simulink model "UPQC_model"  (R2020b)
settings: Solver=FixedStepAuto  StartTime=0.0  StopTime=Tsim  FixedStep=Tsample  MaxStep=Tsample  RelTol=1e-3
values from neighbouring files (symbols this model uses):
  C_parallel_Series = zeros(1,4)    [Netzmodell_Ini_DL.m]    (also in workspace_Ini.mat = [1e-05 1e-05 1e-05 0])
  C_parallel_Shunt = zeros(1,4)    [Netzmodell_Ini_DL.m]    (also in workspace_Ini.mat = [1e-05 1e-05 1e-05 0])
  CC_Ki = 5    [Netzmodell_Ini_DL.m]    (also in workspace_Ini.mat)
  CC_Ki_geg = 5    [Netzmodell_Ini_DL.m]    (also in workspace_Ini.mat)
  CC_Kp = 10    [Netzmodell_Ini_DL.m]    (also in workspace_Ini.mat)
  CC_Kp_geg = 10    [Netzmodell_Ini_DL.m]    (also in workspace_Ini.mat)
  CC_OS =     [workspace_Ini.mat]
  Czk = Szenario.Czk*u    [Netzmodell_Ini_DL.m]    (also in workspace_Ini.mat = 0.003)
  fak_RVC = Szenario.fak_RVC    [Netzmodell_Ini_DL.m]    (also in workspace_Ini.mat = [1 1 1])
  fak_Uns = [1; 1; 1]    [Netzmodell_Ini_DL.m]    (also in workspace_Ini.mat = [1 1 1])
  Flicker_Schaltzeitpunkte_L1 = Schaltzeitpunkte(1,:)    [Netzmodell_Ini_DL.m]    (also in workspace_Ini.mat = 10.5)
  Flicker_Schaltzeitpunkte_L2 = Schaltzeitpunkte(2,:)    [Netzmodell_Ini_DL.m]    (also in workspace_Ini.mat = 10.5)
  Flicker_Schaltzeitpunkte_L3 = Schaltzeitpunkte(3,:)    [Netzmodell_Ini_DL.m]    (also in workspace_Ini.mat = 10.5)
  fs = [f_nom; f_nom; f_nom]    [Netzmodell_Ini_DL.m]    (also in workspace_Ini.mat = [50 50 50])
  fsw = Szenario.fsw*k    [Netzmodell_Ini_DL.m]    (also in workspace_Ini.mat = 20000)
  I_Basis_Ober_L1 = I_Basis_Ober(1)    [Netzmodell_Ini_DL.m]    (also in workspace_Ini.mat = 0)
  I_Basis_Ober_L2 = I_Basis_Ober(2)    [Netzmodell_Ini_DL.m]    (also in workspace_Ini.mat = 0)
  I_Basis_Ober_L3 = I_Basis_Ober(3)    [Netzmodell_Ini_DL.m]    (also in workspace_Ini.mat = 0)
  I_relativ_Ober_L1 = Szenario.I_relativ_Ober_L1    [Netzmodell_Ini_DL.m]    (also in workspace_Ini.mat = [0 100 0 100 100 0 100 100 0 0 0 0 ... (50 elements, 1x50)])
  I_relativ_Ober_L2 = Szenario.I_relativ_Ober_L2    [Netzmodell_Ini_DL.m]    (also in workspace_Ini.mat = [0 100 0 100 100 0 100 100 0 0 0 0 ... (50 elements, 1x50)])
  I_relativ_Ober_L3 = Szenario.I_relativ_Ober_L3    [Netzmodell_Ini_DL.m]    (also in workspace_Ini.mat = [0 100 0 100 100 0 100 100 0 0 0 0 ... (50 elements, 1x50)])
  L_Ausgang_Series = zeros(1,4)    [Netzmodell_Ini_DL.m]    (also in workspace_Ini.mat = [0.00093 0.00093 0.00093 0.00093])
  L_Ausgang_Shunt = zeros(1,4)    [Netzmodell_Ini_DL.m]    (also in workspace_Ini.mat = [0.00093 0.00093 0.00093 0.00093])
  L_Eingang_Series = zeros(1,4)    [Netzmodell_Ini_DL.m]    (also in workspace_Ini.mat = [0.00085 0.00085 0.00085 0.00085])
  L_Eingang_Shunt = zeros(1,4)    [Netzmodell_Ini_DL.m]    (also in workspace_Ini.mat = [0.00085 0.00085 0.00085 0.00085])
  Ls_in = 52.2*u/10    (= 5.22e-06)    [Netzmodell_Ini_DL.m]    (also in workspace_Ini.mat)
  Ltrans = Szenario.Ltrans*m    [Netzmodell_Ini_DL.m]    (also in workspace_Ini.mat = 0.000256)
  OS_off = 6    [Netzmodell_Ini_DL.m]    (also in workspace_Ini.mat)
  OS_on = 1    [Netzmodell_Ini_DL.m]    (also in workspace_Ini.mat)
  Phi_Ober_L1 = Phi_Ober(1)    [Netzmodell_Ini_DL.m]    (also in workspace_Ini.mat = 0)
  Phi_Ober_L2 = Phi_Ober(2)    [Netzmodell_Ini_DL.m]    (also in workspace_Ini.mat = -120)
  Phi_Ober_L3 = Phi_Ober(3)    [Netzmodell_Ini_DL.m]    (also in workspace_Ini.mat = 120)
  Phis = [0; -120; 120]    [Netzmodell_Ini_DL.m]    (also in workspace_Ini.mat = [0 -120 120])
  Pl_Flicker = Pl_Flicker*k    [Netzmodell_Ini_DL.m]    (also in workspace_Ini.mat = [5000 5000 5000])
  Pl_Grund = Szenario.Pl_Grund *k    [Netzmodell_Ini_DL.m]    (also in workspace_Ini.mat = [5 5 5])
  Pl_RVC = Pl_RVC*k    [Netzmodell_Ini_DL.m]    (also in workspace_Ini.mat = [10000 10000 10000])
  Pl_Uns = Pl_Uns*k    [Netzmodell_Ini_DL.m]    (also in workspace_Ini.mat = [25000 10 10])
  Ql_ind_Flicker = Ql_ind_Flicker*k    [Netzmodell_Ini_DL.m]    (also in workspace_Ini.mat = [0 0 0])
  Ql_ind_Grund = Szenario.Ql_ind_Grund*k    [Netzmodell_Ini_DL.m]    (also in workspace_Ini.mat = [0 0 0])
  Ql_ind_RVC = Szenario.Ql_ind_RVC*k    [Netzmodell_Ini_DL.m]    (also in workspace_Ini.mat = [0 0 0])
  Ql_ind_Uns = Ql_ind_Uns*k    [Netzmodell_Ini_DL.m]    (also in workspace_Ini.mat = [0 0 0])
  Ql_kap_Flicker = Ql_kap_Flicker*k    [Netzmodell_Ini_DL.m]    (also in workspace_Ini.mat = [0 0 0])
  Ql_kap_Grund = Szenario.Ql_kap_Grund*k    [Netzmodell_Ini_DL.m]    (also in workspace_Ini.mat = [0 0 0])
  Ql_kap_RVC = Szenario.Ql_kap_RVC*k    [Netzmodell_Ini_DL.m]    (also in workspace_Ini.mat = [0 0 0])
  Ql_kap_Uns = Ql_kap_Uns*k    [Netzmodell_Ini_DL.m]    (also in workspace_Ini.mat = [0 0 0])
  R_Ausgang_Series = zeros(1,4)    [Netzmodell_Ini_DL.m]    (also in workspace_Ini.mat = [0.1 0.1 0.1 0.1])
  R_Ausgang_Shunt = zeros(1,4)    [Netzmodell_Ini_DL.m]    (also in workspace_Ini.mat = [0.1 0.1 0.1 0.1])
  R_Eingang_Series = zeros(1,4)    [Netzmodell_Ini_DL.m]    (also in workspace_Ini.mat = [0.1 0.1 0.1 0.1])
  R_Eingang_Shunt = zeros(1,4)    [Netzmodell_Ini_DL.m]    (also in workspace_Ini.mat = [0.1 0.1 0.1 0.1])
  R_parallel_Series = zeros(1,4)    [Netzmodell_Ini_DL.m]    (also in workspace_Ini.mat = [13 13 13 0])
  R_parallel_Shunt = zeros(1,4)    [Netzmodell_Ini_DL.m]    (also in workspace_Ini.mat = [13 13 13 0])
  R_ZK_Belastung = 20    [Netzmodell_Ini_DL.m]    (also in workspace_Ini.mat)
  Rs_in = 5.2*m/10    (= 0.00052)    [Netzmodell_Ini_DL.m]    (also in workspace_Ini.mat)
  Rtrans = Szenario.Rtrans    [Netzmodell_Ini_DL.m]    (also in workspace_Ini.mat = 0.206)
  RVC_L1_on_off_Zeitpunkte = Szenario.RVC_L1_on_off_Zeitpunkte    [Netzmodell_Ini_DL.m]    (also in workspace_Ini.mat = [10.5 40 10 11 12 13 14 15])
  RVC_L2_on_off_Zeitpunkte = Szenario.RVC_L2_on_off_Zeitpunkte    [Netzmodell_Ini_DL.m]    (also in workspace_Ini.mat = [10.5 40 10 11 12 13 14 15])
  RVC_L3_on_off_Zeitpunkte = Szenario.RVC_L3_on_off_Zeitpunkte    [Netzmodell_Ini_DL.m]    (also in workspace_Ini.mat = [10.5 40 10 11 12 13 14 15])
  RVC_off = 20.5    [Netzmodell_Ini_DL.m]    (also in workspace_Ini.mat)
  RVC_on = 20    [Netzmodell_Ini_DL.m]    (also in workspace_Ini.mat)
  RVC_val = [0.8,0.8,0.8]    [Netzmodell_Ini_DL.m]    (also in workspace_Ini.mat = [0.8 0.8 0.8])
  strans = Szenario.strans    [Netzmodell_Ini_DL.m]    (also in workspace_Ini.mat = 0.25)
  t_breaker_series = tacts    [Netzmodell_Ini_DL.m]    (also in workspace_Ini.mat = 0.5)
  tact = Szenario.tact    [Netzmodell_Ini_DL.m]    (also in workspace_Ini.mat = 0.5)
  tact_OS_Regler = Szenario.tact_OS_Regler    [Netzmodell_Ini_DL.m]    (also in workspace_Ini.mat = 0.5)
  tact_QU = 10    [Netzmodell_Ini_DL.m]    (also in workspace_Ini.mat)
  tacts = Szenario.tacts    [Netzmodell_Ini_DL.m]    (also in workspace_Ini.mat = 0.5)
  Tsample = Szenario.Tsample    [Netzmodell_Ini_DL.m]    (also in workspace_Ini.mat = 5e-06)
  Uns_L1_on_off_Zeitpunkte = Szenario.Uns_L1_on_off_Zeitpunkte    [Netzmodell_Ini_DL.m]    (also in workspace_Ini.mat = [1 6 10 11 12 13 14 15])
  Uns_L2_on_off_Zeitpunkte = Szenario.Uns_L2_on_off_Zeitpunkte    [Netzmodell_Ini_DL.m]    (also in workspace_Ini.mat = [10 30 10 11 12 13 14 15])
  Uns_L3_on_off_Zeitpunkte = Szenario.Uns_L3_on_off_Zeitpunkte    [Netzmodell_Ini_DL.m]    (also in workspace_Ini.mat = [10 30 10 11 12 13 14 15])
  Us = [Us_Amp; Us_Amp; Us_Amp]    [Netzmodell_Ini_DL.m]    (also in workspace_Ini.mat = [326.598632371 326.598632371 326.598632371])
  Us_Amp = sqrt(2)*400/sqrt(3)    [Netzmodell_Ini_DL.m]    (also in workspace_Ini.mat = 326.598632371)
  VC_Ki_gegen = 30    [Netzmodell_Ini_DL.m]    (also in workspace_Ini.mat)
  VC_Ki_gegen_shunt = 15    [Netzmodell_Ini_DL.m]    (also in workspace_Ini.mat)
  VC_Ki_mit = 5    [Netzmodell_Ini_DL.m]    (also in workspace_Ini.mat)
  VC_Kp_gegen = 5    [workspace_Ini.mat]
  VC_Kp_gegen_shunt = 2    [Netzmodell_Ini_DL.m]    (also in workspace_Ini.mat)
  VC_Kp_mit = 10    [Netzmodell_Ini_DL.m]    (also in workspace_Ini.mat)
  VC_ZK_Ki = 5    [Netzmodell_Ini_DL.m]    (also in workspace_Ini.mat)
  VC_ZK_Kp = 0.5    [Netzmodell_Ini_DL.m]    (also in workspace_Ini.mat)
  Vielfache_Ober_L1 = Szenario.Vielfache_Ober_L1    [Netzmodell_Ini_DL.m]    (also in workspace_Ini.mat = [1 2 3 4 5 6 7 8 9 10 11 12 ... (50 elements, 1x50)])
  Vielfache_Ober_L2 = Szenario.Vielfache_Ober_L2    [Netzmodell_Ini_DL.m]    (also in workspace_Ini.mat = [1 2 3 4 5 6 7 8 9 10 11 12 ... (50 elements, 1x50)])
  Vielfache_Ober_L3 = Szenario.Vielfache_Ober_L3    [Netzmodell_Ini_DL.m]    (also in workspace_Ini.mat = [1 2 3 4 5 6 7 8 9 10 11 12 ... (50 elements, 1x50)])
  ZK_Belastung_off = 100    [Netzmodell_Ini_DL.m]    (also in workspace_Ini.mat)
  ZK_Belastung_on = 100    [Netzmodell_Ini_DL.m]    (also in workspace_Ini.mat)
  Zwischenkreisspannung = 700    [Netzmodell_Ini_DL.m]    (also in workspace_Ini.mat)
undefined symbols (not defined in the file or in its folder): LAusgang, RReiheL3
libraries: powerlib x221, powerlib_meascontrol x80, pid_lib x23, eeTransforms x4, eePwmGeneratorTwoLevel x2, dspstat3 x1
(part 11 of 16)

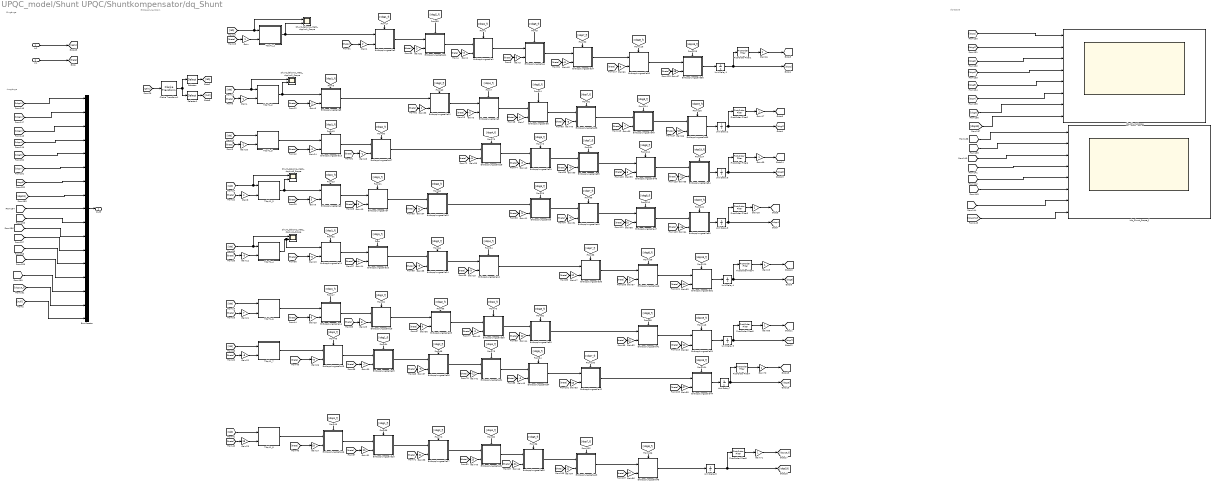
== system UPQC_model/Shunt UPQC/Shuntkompensator/dq_Shunt ==
  note: Entkopplung Strom
  note: Eingänge
  note: Ausgänge
  note: dq-Scope
  In2 : Inport
  In1 : Inport  Port=2
  Bus Creator : BusCreator  Inputs=17
  Clarke Transform1 : eeTransforms/Clarke Transform  PowerInvariant=off
      settings: SourceProductBaseCode=PS
  Entkopplungszelle1 : Subsystem
      settings: PortSchema="{\"entries\":[{\"content\":{\"sides\":[{\"content\":{\"connectorIds\":[\"In1\",\"In2\"]},\"type\":\"ConnectorPlacement.EquallySpacedRectSide\",\"uuid\":\"e8e24803-2fc0-483c-82f9-6ee33f65ebd9\"},{\"content\":{\"connectorIds\":[\"Out1\"],\"side\":\"RIGHT\"},\"type\":\"ConnectorPlacement.EquallySpacedRectSide\",\"uuid\":\"e11e5831-ab5e-42bb-bd0b-63825273f403\"},{\"content\":{\"connectorIds\":[\"In3\"],\"side\":\"TOP\"},\"type\":\"ConnectorPlacement.EquallySpacedRectSide\",\"uuid\":\"2b39bd07-2b6e-4e89-bb54-1321cea2c793\"},{\"content\":{\"connectorIds\":[],\"side\":\"HIDDEN\"},\"type\":\"ConnectorPlacement.EquallySpacedRectSide\",\"uuid\":\"a99c5943-5af0-4d11-8875-695bd24f17f4\"}]},\"type\":\"ConnectorPlacement.EquallySpacedConnector\",\"uuid\":\"a2a714db-f067-4e0e-8919-f68d1dab84ba\"}],\"packageUris\":[\"http://schema.mathworks.com/mf0/Connector/R2020b\"],\"version\":\"1.0\"}"
  Entkopplungszelle10 : Subsystem
      settings: PortSchema="{\"entries\":[{\"content\":{\"sides\":[{\"content\":{\"connectorIds\":[\"In1\",\"In2\"]},\"type\":\"ConnectorPlacement.EquallySpacedRectSide\",\"uuid\":\"e8e24803-2fc0-483c-82f9-6ee33f65ebd9\"},{\"content\":{\"connectorIds\":[\"Out1\"],\"side\":\"RIGHT\"},\"type\":\"ConnectorPlacement.EquallySpacedRectSide\",\"uuid\":\"e11e5831-ab5e-42bb-bd0b-63825273f403\"},{\"content\":{\"connectorIds\":[\"In3\"],\"side\":\"TOP\"},\"type\":\"ConnectorPlacement.EquallySpacedRectSide\",\"uuid\":\"2b39bd07-2b6e-4e89-bb54-1321cea2c793\"},{\"content\":{\"connectorIds\":[],\"side\":\"HIDDEN\"},\"type\":\"ConnectorPlacement.EquallySpacedRectSide\",\"uuid\":\"a99c5943-5af0-4d11-8875-695bd24f17f4\"}]},\"type\":\"ConnectorPlacement.EquallySpacedConnector\",\"uuid\":\"a2a714db-f067-4e0e-8919-f68d1dab84ba\"}],\"packageUris\":[\"http://schema.mathworks.com/mf0/Connector/R2020b\"],\"version\":\"1.0\"}"
  Entkopplungszelle11 : Subsystem
      settings: PortSchema="{\"entries\":[{\"content\":{\"sides\":[{\"content\":{\"connectorIds\":[\"In1\",\"In2\"]},\"type\":\"ConnectorPlacement.EquallySpacedRectSide\",\"uuid\":\"e8e24803-2fc0-483c-82f9-6ee33f65ebd9\"},{\"content\":{\"connectorIds\":[\"Out1\"],\"side\":\"RIGHT\"},\"type\":\"ConnectorPlacement.EquallySpacedRectSide\",\"uuid\":\"e11e5831-ab5e-42bb-bd0b-63825273f403\"},{\"content\":{\"connectorIds\":[\"In3\"],\"side\":\"TOP\"},\"type\":\"ConnectorPlacement.EquallySpacedRectSide\",\"uuid\":\"2b39bd07-2b6e-4e89-bb54-1321cea2c793\"},{\"content\":{\"connectorIds\":[],\"side\":\"HIDDEN\"},\"type\":\"ConnectorPlacement.EquallySpacedRectSide\",\"uuid\":\"a99c5943-5af0-4d11-8875-695bd24f17f4\"}]},\"type\":\"ConnectorPlacement.EquallySpacedConnector\",\"uuid\":\"a2a714db-f067-4e0e-8919-f68d1dab84ba\"}],\"packageUris\":[\"http://schema.mathworks.com/mf0/Connector/R2020b\"],\"version\":\"1.0\"}"
  Entkopplungszelle12 : Subsystem
      settings: PortSchema="{\"entries\":[{\"content\":{\"sides\":[{\"content\":{\"connectorIds\":[\"In1\",\"In2\"]},\"type\":\"ConnectorPlacement.EquallySpacedRectSide\",\"uuid\":\"e8e24803-2fc0-483c-82f9-6ee33f65ebd9\"},{\"content\":{\"connectorIds\":[\"Out1\"],\"side\":\"RIGHT\"},\"type\":\"ConnectorPlacement.EquallySpacedRectSide\",\"uuid\":\"e11e5831-ab5e-42bb-bd0b-63825273f403\"},{\"content\":{\"connectorIds\":[\"In3\"],\"side\":\"TOP\"},\"type\":\"ConnectorPlacement.EquallySpacedRectSide\",\"uuid\":\"2b39bd07-2b6e-4e89-bb54-1321cea2c793\"},{\"content\":{\"connectorIds\":[],\"side\":\"HIDDEN\"},\"type\":\"ConnectorPlacement.EquallySpacedRectSide\",\"uuid\":\"a99c5943-5af0-4d11-8875-695bd24f17f4\"}]},\"type\":\"ConnectorPlacement.EquallySpacedConnector\",\"uuid\":\"a2a714db-f067-4e0e-8919-f68d1dab84ba\"}],\"packageUris\":[\"http://schema.mathworks.com/mf0/Connector/R2020b\"],\"version\":\"1.0\"}"
  Entkopplungszelle13 : Subsystem
      settings: PortSchema="{\"entries\":[{\"content\":{\"sides\":[{\"content\":{\"connectorIds\":[\"In1\",\"In2\"]},\"type\":\"ConnectorPlacement.EquallySpacedRectSide\",\"uuid\":\"e8e24803-2fc0-483c-82f9-6ee33f65ebd9\"},{\"content\":{\"connectorIds\":[\"Out1\"],\"side\":\"RIGHT\"},\"type\":\"ConnectorPlacement.EquallySpacedRectSide\",\"uuid\":\"e11e5831-ab5e-42bb-bd0b-63825273f403\"},{\"content\":{\"connectorIds\":[\"In3\"],\"side\":\"TOP\"},\"type\":\"ConnectorPlacement.EquallySpacedRectSide\",\"uuid\":\"2b39bd07-2b6e-4e89-bb54-1321cea2c793\"},{\"content\":{\"connectorIds\":[],\"side\":\"HIDDEN\"},\"type\":\"ConnectorPlacement.EquallySpacedRectSide\",\"uuid\":\"a99c5943-5af0-4d11-8875-695bd24f17f4\"}]},\"type\":\"ConnectorPlacement.EquallySpacedConnector\",\"uuid\":\"a2a714db-f067-4e0e-8919-f68d1dab84ba\"}],\"packageUris\":[\"http://schema.mathworks.com/mf0/Connector/R2020b\"],\"version\":\"1.0\"}"
  Entkopplungszelle14 : Subsystem
      settings: PortSchema="{\"entries\":[{\"content\":{\"sides\":[{\"content\":{\"connectorIds\":[\"In1\",\"In2\"]},\"type\":\"ConnectorPlacement.EquallySpacedRectSide\",\"uuid\":\"e8e24803-2fc0-483c-82f9-6ee33f65ebd9\"},{\"content\":{\"connectorIds\":[\"Out1\"],\"side\":\"RIGHT\"},\"type\":\"ConnectorPlacement.EquallySpacedRectSide\",\"uuid\":\"e11e5831-ab5e-42bb-bd0b-63825273f403\"},{\"content\":{\"connectorIds\":[\"In3\"],\"side\":\"TOP\"},\"type\":\"ConnectorPlacement.EquallySpacedRectSide\",\"uuid\":\"2b39bd07-2b6e-4e89-bb54-1321cea2c793\"},{\"content\":{\"connectorIds\":[],\"side\":\"HIDDEN\"},\"type\":\"ConnectorPlacement.EquallySpacedRectSide\",\"uuid\":\"a99c5943-5af0-4d11-8875-695bd24f17f4\"}]},\"type\":\"ConnectorPlacement.EquallySpacedConnector\",\"uuid\":\"a2a714db-f067-4e0e-8919-f68d1dab84ba\"}],\"packageUris\":[\"http://schema.mathworks.com/mf0/Connector/R2020b\"],\"version\":\"1.0\"}"
  Entkopplungszelle15 : Subsystem
      settings: PortSchema="{\"entries\":[{\"content\":{\"sides\":[{\"content\":{\"connectorIds\":[\"In1\",\"In2\"]},\"type\":\"ConnectorPlacement.EquallySpacedRectSide\",\"uuid\":\"e8e24803-2fc0-483c-82f9-6ee33f65ebd9\"},{\"content\":{\"connectorIds\":[\"Out1\"],\"side\":\"RIGHT\"},\"type\":\"ConnectorPlacement.EquallySpacedRectSide\",\"uuid\":\"e11e5831-ab5e-42bb-bd0b-63825273f403\"},{\"content\":{\"connectorIds\":[\"In3\"],\"side\":\"TOP\"},\"type\":\"ConnectorPlacement.EquallySpacedRectSide\",\"uuid\":\"2b39bd07-2b6e-4e89-bb54-1321cea2c793\"},{\"content\":{\"connectorIds\":[],\"side\":\"HIDDEN\"},\"type\":\"ConnectorPlacement.EquallySpacedRectSide\",\"uuid\":\"a99c5943-5af0-4d11-8875-695bd24f17f4\"}]},\"type\":\"ConnectorPlacement.EquallySpacedConnector\",\"uuid\":\"a2a714db-f067-4e0e-8919-f68d1dab84ba\"}],\"packageUris\":[\"http://schema.mathworks.com/mf0/Connector/R2020b\"],\"version\":\"1.0\"}"
  Entkopplungszelle16 : Subsystem
      settings: PortSchema="{\"entries\":[{\"content\":{\"sides\":[{\"content\":{\"connectorIds\":[\"In1\",\"In2\"]},\"type\":\"ConnectorPlacement.EquallySpacedRectSide\",\"uuid\":\"e8e24803-2fc0-483c-82f9-6ee33f65ebd9\"},{\"content\":{\"connectorIds\":[\"Out1\"],\"side\":\"RIGHT\"},\"type\":\"ConnectorPlacement.EquallySpacedRectSide\",\"uuid\":\"e11e5831-ab5e-42bb-bd0b-63825273f403\"},{\"content\":{\"connectorIds\":[\"In3\"],\"side\":\"TOP\"},\"type\":\"ConnectorPlacement.EquallySpacedRectSide\",\"uuid\":\"2b39bd07-2b6e-4e89-bb54-1321cea2c793\"},{\"content\":{\"connectorIds\":[],\"side\":\"HIDDEN\"},\"type\":\"ConnectorPlacement.EquallySpacedRectSide\",\"uuid\":\"a99c5943-5af0-4d11-8875-695bd24f17f4\"}]},\"type\":\"ConnectorPlacement.EquallySpacedConnector\",\"uuid\":\"a2a714db-f067-4e0e-8919-f68d1dab84ba\"}],\"packageUris\":[\"http://schema.mathworks.com/mf0/Connector/R2020b\"],\"version\":\"1.0\"}"
  Entkopplungszelle17 : Subsystem
      settings: PortSchema="{\"entries\":[{\"content\":{\"sides\":[{\"content\":{\"connectorIds\":[\"In1\",\"In2\"]},\"type\":\"ConnectorPlacement.EquallySpacedRectSide\",\"uuid\":\"e8e24803-2fc0-483c-82f9-6ee33f65ebd9\"},{\"content\":{\"connectorIds\":[\"Out1\"],\"side\":\"RIGHT\"},\"type\":\"ConnectorPlacement.EquallySpacedRectSide\",\"uuid\":\"e11e5831-ab5e-42bb-bd0b-63825273f403\"},{\"content\":{\"connectorIds\":[\"In3\"],\"side\":\"TOP\"},\"type\":\"ConnectorPlacement.EquallySpacedRectSide\",\"uuid\":\"2b39bd07-2b6e-4e89-bb54-1321cea2c793\"},{\"content\":{\"connectorIds\":[],\"side\":\"HIDDEN\"},\"type\":\"ConnectorPlacement.EquallySpacedRectSide\",\"uuid\":\"a99c5943-5af0-4d11-8875-695bd24f17f4\"}]},\"type\":\"ConnectorPlacement.EquallySpacedConnector\",\"uuid\":\"a2a714db-f067-4e0e-8919-f68d1dab84ba\"}],\"packageUris\":[\"http://schema.mathworks.com/mf0/Connector/R2020b\"],\"version\":\"1.0\"}"
  Entkopplungszelle18 : Subsystem
      settings: PortSchema="{\"entries\":[{\"content\":{\"sides\":[{\"content\":{\"connectorIds\":[\"In1\",\"In2\"]},\"type\":\"ConnectorPlacement.EquallySpacedRectSide\",\"uuid\":\"e8e24803-2fc0-483c-82f9-6ee33f65ebd9\"},{\"content\":{\"connectorIds\":[\"Out1\"],\"side\":\"RIGHT\"},\"type\":\"ConnectorPlacement.EquallySpacedRectSide\",\"uuid\":\"e11e5831-ab5e-42bb-bd0b-63825273f403\"},{\"content\":{\"connectorIds\":[\"In3\"],\"side\":\"TOP\"},\"type\":\"ConnectorPlacement.EquallySpacedRectSide\",\"uuid\":\"2b39bd07-2b6e-4e89-bb54-1321cea2c793\"},{\"content\":{\"connectorIds\":[],\"side\":\"HIDDEN\"},\"type\":\"ConnectorPlacement.EquallySpacedRectSide\",\"uuid\":\"a99c5943-5af0-4d11-8875-695bd24f17f4\"}]},\"type\":\"ConnectorPlacement.EquallySpacedConnector\",\"uuid\":\"a2a714db-f067-4e0e-8919-f68d1dab84ba\"}],\"packageUris\":[\"http://schema.mathworks.com/mf0/Connector/R2020b\"],\"version\":\"1.0\"}"
  Entkopplungszelle19 : Subsystem
      settings: PortSchema="{\"entries\":[{\"content\":{\"sides\":[{\"content\":{\"connectorIds\":[\"In1\",\"In2\"]},\"type\":\"ConnectorPlacement.EquallySpacedRectSide\",\"uuid\":\"e8e24803-2fc0-483c-82f9-6ee33f65ebd9\"},{\"content\":{\"connectorIds\":[\"Out1\"],\"side\":\"RIGHT\"},\"type\":\"ConnectorPlacement.EquallySpacedRectSide\",\"uuid\":\"e11e5831-ab5e-42bb-bd0b-63825273f403\"},{\"content\":{\"connectorIds\":[\"In3\"],\"side\":\"TOP\"},\"type\":\"ConnectorPlacement.EquallySpacedRectSide\",\"uuid\":\"2b39bd07-2b6e-4e89-bb54-1321cea2c793\"},{\"content\":{\"connectorIds\":[],\"side\":\"HIDDEN\"},\"type\":\"ConnectorPlacement.EquallySpacedRectSide\",\"uuid\":\"a99c5943-5af0-4d11-8875-695bd24f17f4\"}]},\"type\":\"ConnectorPlacement.EquallySpacedConnector\",\"uuid\":\"a2a714db-f067-4e0e-8919-f68d1dab84ba\"}],\"packageUris\":[\"http://schema.mathworks.com/mf0/Connector/R2020b\"],\"version\":\"1.0\"}"
  Entkopplungszelle2 : Subsystem
      settings: PortSchema="{\"entries\":[{\"content\":{\"sides\":[{\"content\":{\"connectorIds\":[\"In1\",\"In2\"]},\"type\":\"ConnectorPlacement.EquallySpacedRectSide\",\"uuid\":\"e8e24803-2fc0-483c-82f9-6ee33f65ebd9\"},{\"content\":{\"connectorIds\":[\"Out1\"],\"side\":\"RIGHT\"},\"type\":\"ConnectorPlacement.EquallySpacedRectSide\",\"uuid\":\"e11e5831-ab5e-42bb-bd0b-63825273f403\"},{\"content\":{\"connectorIds\":[\"In3\"],\"side\":\"TOP\"},\"type\":\"ConnectorPlacement.EquallySpacedRectSide\",\"uuid\":\"2b39bd07-2b6e-4e89-bb54-1321cea2c793\"},{\"content\":{\"connectorIds\":[],\"side\":\"HIDDEN\"},\"type\":\"ConnectorPlacement.EquallySpacedRectSide\",\"uuid\":\"a99c5943-5af0-4d11-8875-695bd24f17f4\"}]},\"type\":\"ConnectorPlacement.EquallySpacedConnector\",\"uuid\":\"a2a714db-f067-4e0e-8919-f68d1dab84ba\"}],\"packageUris\":[\"http://schema.mathworks.com/mf0/Connector/R2020b\"],\"version\":\"1.0\"}"
  Entkopplungszelle20 : Subsystem
      settings: PortSchema="{\"entries\":[{\"content\":{\"sides\":[{\"content\":{\"connectorIds\":[\"In1\",\"In2\"]},\"type\":\"ConnectorPlacement.EquallySpacedRectSide\",\"uuid\":\"e8e24803-2fc0-483c-82f9-6ee33f65ebd9\"},{\"content\":{\"connectorIds\":[\"Out1\"],\"side\":\"RIGHT\"},\"type\":\"ConnectorPlacement.EquallySpacedRectSide\",\"uuid\":\"e11e5831-ab5e-42bb-bd0b-63825273f403\"},{\"content\":{\"connectorIds\":[\"In3\"],\"side\":\"TOP\"},\"type\":\"ConnectorPlacement.EquallySpacedRectSide\",\"uuid\":\"2b39bd07-2b6e-4e89-bb54-1321cea2c793\"},{\"content\":{\"connectorIds\":[],\"side\":\"HIDDEN\"},\"type\":\"ConnectorPlacement.EquallySpacedRectSide\",\"uuid\":\"a99c5943-5af0-4d11-8875-695bd24f17f4\"}]},\"type\":\"ConnectorPlacement.EquallySpacedConnector\",\"uuid\":\"a2a714db-f067-4e0e-8919-f68d1dab84ba\"}],\"packageUris\":[\"http://schema.mathworks.com/mf0/Connector/R2020b\"],\"version\":\"1.0\"}"
  Entkopplungszelle21 : Subsystem
      settings: PortSchema="{\"entries\":[{\"content\":{\"sides\":[{\"content\":{\"connectorIds\":[\"In1\",\"In2\"]},\"type\":\"ConnectorPlacement.EquallySpacedRectSide\",\"uuid\":\"e8e24803-2fc0-483c-82f9-6ee33f65ebd9\"},{\"content\":{\"connectorIds\":[\"Out1\"],\"side\":\"RIGHT\"},\"type\":\"ConnectorPlacement.EquallySpacedRectSide\",\"uuid\":\"e11e5831-ab5e-42bb-bd0b-63825273f403\"},{\"content\":{\"connectorIds\":[\"In3\"],\"side\":\"TOP\"},\"type\":\"ConnectorPlacement.EquallySpacedRectSide\",\"uuid\":\"2b39bd07-2b6e-4e89-bb54-1321cea2c793\"},{\"content\":{\"connectorIds\":[],\"side\":\"HIDDEN\"},\"type\":\"ConnectorPlacement.EquallySpacedRectSide\",\"uuid\":\"a99c5943-5af0-4d11-8875-695bd24f17f4\"}]},\"type\":\"ConnectorPlacement.EquallySpacedConnector\",\"uuid\":\"a2a714db-f067-4e0e-8919-f68d1dab84ba\"}],\"packageUris\":[\"http://schema.mathworks.com/mf0/Connector/R2020b\"],\"version\":\"1.0\"}"
  Entkopplungszelle22 : Subsystem
      settings: PortSchema="{\"entries\":[{\"content\":{\"sides\":[{\"content\":{\"connectorIds\":[\"In1\",\"In2\"]},\"type\":\"ConnectorPlacement.EquallySpacedRectSide\",\"uuid\":\"e8e24803-2fc0-483c-82f9-6ee33f65ebd9\"},{\"content\":{\"connectorIds\":[\"Out1\"],\"side\":\"RIGHT\"},\"type\":\"ConnectorPlacement.EquallySpacedRectSide\",\"uuid\":\"e11e5831-ab5e-42bb-bd0b-63825273f403\"},{\"content\":{\"connectorIds\":[\"In3\"],\"side\":\"TOP\"},\"type\":\"ConnectorPlacement.EquallySpacedRectSide\",\"uuid\":\"2b39bd07-2b6e-4e89-bb54-1321cea2c793\"},{\"content\":{\"connectorIds\":[],\"side\":\"HIDDEN\"},\"type\":\"ConnectorPlacement.EquallySpacedRectSide\",\"uuid\":\"a99c5943-5af0-4d11-8875-695bd24f17f4\"}]},\"type\":\"ConnectorPlacement.EquallySpacedConnector\",\"uuid\":\"a2a714db-f067-4e0e-8919-f68d1dab84ba\"}],\"packageUris\":[\"http://schema.mathworks.com/mf0/Connector/R2020b\"],\"version\":\"1.0\"}"
  Entkopplungszelle23 : Subsystem
      settings: PortSchema="{\"entries\":[{\"content\":{\"sides\":[{\"content\":{\"connectorIds\":[\"In1\",\"In2\"]},\"type\":\"ConnectorPlacement.EquallySpacedRectSide\",\"uuid\":\"e8e24803-2fc0-483c-82f9-6ee33f65ebd9\"},{\"content\":{\"connectorIds\":[\"Out1\"],\"side\":\"RIGHT\"},\"type\":\"ConnectorPlacement.EquallySpacedRectSide\",\"uuid\":\"e11e5831-ab5e-42bb-bd0b-63825273f403\"},{\"content\":{\"connectorIds\":[\"In3\"],\"side\":\"TOP\"},\"type\":\"ConnectorPlacement.EquallySpacedRectSide\",\"uuid\":\"2b39bd07-2b6e-4e89-bb54-1321cea2c793\"},{\"content\":{\"connectorIds\":[],\"side\":\"HIDDEN\"},\"type\":\"ConnectorPlacement.EquallySpacedRectSide\",\"uuid\":\"a99c5943-5af0-4d11-8875-695bd24f17f4\"}]},\"type\":\"ConnectorPlacement.EquallySpacedConnector\",\"uuid\":\"a2a714db-f067-4e0e-8919-f68d1dab84ba\"}],\"packageUris\":[\"http://schema.mathworks.com/mf0/Connector/R2020b\"],\"version\":\"1.0\"}"
  Entkopplungszelle24 : Subsystem
      settings: PortSchema="{\"entries\":[{\"content\":{\"sides\":[{\"content\":{\"connectorIds\":[\"In1\",\"In2\"]},\"type\":\"ConnectorPlacement.EquallySpacedRectSide\",\"uuid\":\"e8e24803-2fc0-483c-82f9-6ee33f65ebd9\"},{\"content\":{\"connectorIds\":[\"Out1\"],\"side\":\"RIGHT\"},\"type\":\"ConnectorPlacement.EquallySpacedRectSide\",\"uuid\":\"e11e5831-ab5e-42bb-bd0b-63825273f403\"},{\"content\":{\"connectorIds\":[\"In3\"],\"side\":\"TOP\"},\"type\":\"ConnectorPlacement.EquallySpacedRectSide\",\"uuid\":\"2b39bd07-2b6e-4e89-bb54-1321cea2c793\"},{\"content\":{\"connectorIds\":[],\"side\":\"HIDDEN\"},\"type\":\"ConnectorPlacement.EquallySpacedRectSide\",\"uuid\":\"a99c5943-5af0-4d11-8875-695bd24f17f4\"}]},\"type\":\"ConnectorPlacement.EquallySpacedConnector\",\"uuid\":\"a2a714db-f067-4e0e-8919-f68d1dab84ba\"}],\"packageUris\":[\"http://schema.mathworks.com/mf0/Connector/R2020b\"],\"version\":\"1.0\"}"
  Entkopplungszelle25 : Subsystem
      settings: PortSchema="{\"entries\":[{\"content\":{\"sides\":[{\"content\":{\"connectorIds\":[\"In1\",\"In2\"]},\"type\":\"ConnectorPlacement.EquallySpacedRectSide\",\"uuid\":\"e8e24803-2fc0-483c-82f9-6ee33f65ebd9\"},{\"content\":{\"connectorIds\":[\"Out1\"],\"side\":\"RIGHT\"},\"type\":\"ConnectorPlacement.EquallySpacedRectSide\",\"uuid\":\"e11e5831-ab5e-42bb-bd0b-63825273f403\"},{\"content\":{\"connectorIds\":[\"In3\"],\"side\":\"TOP\"},\"type\":\"ConnectorPlacement.EquallySpacedRectSide\",\"uuid\":\"2b39bd07-2b6e-4e89-bb54-1321cea2c793\"},{\"content\":{\"connectorIds\":[],\"side\":\"HIDDEN\"},\"type\":\"ConnectorPlacement.EquallySpacedRectSide\",\"uuid\":\"a99c5943-5af0-4d11-8875-695bd24f17f4\"}]},\"type\":\"ConnectorPlacement.EquallySpacedConnector\",\"uuid\":\"a2a714db-f067-4e0e-8919-f68d1dab84ba\"}],\"packageUris\":[\"http://schema.mathworks.com/mf0/Connector/R2020b\"],\"version\":\"1.0\"}"
  Entkopplungszelle26 : Subsystem
      settings: PortSchema="{\"entries\":[{\"content\":{\"sides\":[{\"content\":{\"connectorIds\":[\"In1\",\"In2\"]},\"type\":\"ConnectorPlacement.EquallySpacedRectSide\",\"uuid\":\"e8e24803-2fc0-483c-82f9-6ee33f65ebd9\"},{\"content\":{\"connectorIds\":[\"Out1\"],\"side\":\"RIGHT\"},\"type\":\"ConnectorPlacement.EquallySpacedRectSide\",\"uuid\":\"e11e5831-ab5e-42bb-bd0b-63825273f403\"},{\"content\":{\"connectorIds\":[\"In3\"],\"side\":\"TOP\"},\"type\":\"ConnectorPlacement.EquallySpacedRectSide\",\"uuid\":\"2b39bd07-2b6e-4e89-bb54-1321cea2c793\"},{\"content\":{\"connectorIds\":[],\"side\":\"HIDDEN\"},\"type\":\"ConnectorPlacement.EquallySpacedRectSide\",\"uuid\":\"a99c5943-5af0-4d11-8875-695bd24f17f4\"}]},\"type\":\"ConnectorPlacement.EquallySpacedConnector\",\"uuid\":\"a2a714db-f067-4e0e-8919-f68d1dab84ba\"}],\"packageUris\":[\"http://schema.mathworks.com/mf0/Connector/R2020b\"],\"version\":\"1.0\"}"
  Entkopplungszelle27 : Subsystem
      settings: PortSchema="{\"entries\":[{\"content\":{\"sides\":[{\"content\":{\"connectorIds\":[\"In1\",\"In2\"]},\"type\":\"ConnectorPlacement.EquallySpacedRectSide\",\"uuid\":\"e8e24803-2fc0-483c-82f9-6ee33f65ebd9\"},{\"content\":{\"connectorIds\":[\"Out1\"],\"side\":\"RIGHT\"},\"type\":\"ConnectorPlacement.EquallySpacedRectSide\",\"uuid\":\"e11e5831-ab5e-42bb-bd0b-63825273f403\"},{\"content\":{\"connectorIds\":[\"In3\"],\"side\":\"TOP\"},\"type\":\"ConnectorPlacement.EquallySpacedRectSide\",\"uuid\":\"2b39bd07-2b6e-4e89-bb54-1321cea2c793\"},{\"content\":{\"connectorIds\":[],\"side\":\"HIDDEN\"},\"type\":\"ConnectorPlacement.EquallySpacedRectSide\",\"uuid\":\"a99c5943-5af0-4d11-8875-695bd24f17f4\"}]},\"type\":\"ConnectorPlacement.EquallySpacedConnector\",\"uuid\":\"a2a714db-f067-4e0e-8919-f68d1dab84ba\"}],\"packageUris\":[\"http://schema.mathworks.com/mf0/Connector/R2020b\"],\"version\":\"1.0\"}"
  Entkopplungszelle28 : Subsystem
      settings: PortSchema="{\"entries\":[{\"content\":{\"sides\":[{\"content\":{\"connectorIds\":[\"In1\",\"In2\"]},\"type\":\"ConnectorPlacement.EquallySpacedRectSide\",\"uuid\":\"e8e24803-2fc0-483c-82f9-6ee33f65ebd9\"},{\"content\":{\"connectorIds\":[\"Out1\"],\"side\":\"RIGHT\"},\"type\":\"ConnectorPlacement.EquallySpacedRectSide\",\"uuid\":\"e11e5831-ab5e-42bb-bd0b-63825273f403\"},{\"content\":{\"connectorIds\":[\"In3\"],\"side\":\"TOP\"},\"type\":\"ConnectorPlacement.EquallySpacedRectSide\",\"uuid\":\"2b39bd07-2b6e-4e89-bb54-1321cea2c793\"},{\"content\":{\"connectorIds\":[],\"side\":\"HIDDEN\"},\"type\":\"ConnectorPlacement.EquallySpacedRectSide\",\"uuid\":\"a99c5943-5af0-4d11-8875-695bd24f17f4\"}]},\"type\":\"ConnectorPlacement.EquallySpacedConnector\",\"uuid\":\"a2a714db-f067-4e0e-8919-f68d1dab84ba\"}],\"packageUris\":[\"http://schema.mathworks.com/mf0/Connector/R2020b\"],\"version\":\"1.0\"}"
  Entkopplungszelle29 : Subsystem
      settings: PortSchema="{\"entries\":[{\"content\":{\"sides\":[{\"content\":{\"connectorIds\":[\"In1\",\"In2\"]},\"type\":\"ConnectorPlacement.EquallySpacedRectSide\",\"uuid\":\"e8e24803-2fc0-483c-82f9-6ee33f65ebd9\"},{\"content\":{\"connectorIds\":[\"Out1\"],\"side\":\"RIGHT\"},\"type\":\"ConnectorPlacement.EquallySpacedRectSide\",\"uuid\":\"e11e5831-ab5e-42bb-bd0b-63825273f403\"},{\"content\":{\"connectorIds\":[\"In3\"],\"side\":\"TOP\"},\"type\":\"ConnectorPlacement.EquallySpacedRectSide\",\"uuid\":\"2b39bd07-2b6e-4e89-bb54-1321cea2c793\"},{\"content\":{\"connectorIds\":[],\"side\":\"HIDDEN\"},\"type\":\"ConnectorPlacement.EquallySpacedRectSide\",\"uuid\":\"a99c5943-5af0-4d11-8875-695bd24f17f4\"}]},\"type\":\"ConnectorPlacement.EquallySpacedConnector\",\"uuid\":\"a2a714db-f067-4e0e-8919-f68d1dab84ba\"}],\"packageUris\":[\"http://schema.mathworks.com/mf0/Connector/R2020b\"],\"version\":\"1.0\"}"
  Entkopplungszelle3 : Subsystem
      settings: PortSchema="{\"entries\":[{\"content\":{\"sides\":[{\"content\":{\"connectorIds\":[\"In1\",\"In2\"]},\"type\":\"ConnectorPlacement.EquallySpacedRectSide\",\"uuid\":\"e8e24803-2fc0-483c-82f9-6ee33f65ebd9\"},{\"content\":{\"connectorIds\":[\"Out1\"],\"side\":\"RIGHT\"},\"type\":\"ConnectorPlacement.EquallySpacedRectSide\",\"uuid\":\"e11e5831-ab5e-42bb-bd0b-63825273f403\"},{\"content\":{\"connectorIds\":[\"In3\"],\"side\":\"TOP\"},\"type\":\"ConnectorPlacement.EquallySpacedRectSide\",\"uuid\":\"2b39bd07-2b6e-4e89-bb54-1321cea2c793\"},{\"content\":{\"connectorIds\":[],\"side\":\"HIDDEN\"},\"type\":\"ConnectorPlacement.EquallySpacedRectSide\",\"uuid\":\"a99c5943-5af0-4d11-8875-695bd24f17f4\"}]},\"type\":\"ConnectorPlacement.EquallySpacedConnector\",\"uuid\":\"a2a714db-f067-4e0e-8919-f68d1dab84ba\"}],\"packageUris\":[\"http://schema.mathworks.com/mf0/Connector/R2020b\"],\"version\":\"1.0\"}"
  Entkopplungszelle30 : Subsystem
      settings: PortSchema="{\"entries\":[{\"content\":{\"sides\":[{\"content\":{\"connectorIds\":[\"In1\",\"In2\"]},\"type\":\"ConnectorPlacement.EquallySpacedRectSide\",\"uuid\":\"e8e24803-2fc0-483c-82f9-6ee33f65ebd9\"},{\"content\":{\"connectorIds\":[\"Out1\"],\"side\":\"RIGHT\"},\"type\":\"ConnectorPlacement.EquallySpacedRectSide\",\"uuid\":\"e11e5831-ab5e-42bb-bd0b-63825273f403\"},{\"content\":{\"connectorIds\":[\"In3\"],\"side\":\"TOP\"},\"type\":\"ConnectorPlacement.EquallySpacedRectSide\",\"uuid\":\"2b39bd07-2b6e-4e89-bb54-1321cea2c793\"},{\"content\":{\"connectorIds\":[],\"side\":\"HIDDEN\"},\"type\":\"ConnectorPlacement.EquallySpacedRectSide\",\"uuid\":\"a99c5943-5af0-4d11-8875-695bd24f17f4\"}]},\"type\":\"ConnectorPlacement.EquallySpacedConnector\",\"uuid\":\"a2a714db-f067-4e0e-8919-f68d1dab84ba\"}],\"packageUris\":[\"http://schema.mathworks.com/mf0/Connector/R2020b\"],\"version\":\"1.0\"}"
  Entkopplungszelle31 : Subsystem
      settings: PortSchema="{\"entries\":[{\"content\":{\"sides\":[{\"content\":{\"connectorIds\":[\"In1\",\"In2\"]},\"type\":\"ConnectorPlacement.EquallySpacedRectSide\",\"uuid\":\"e8e24803-2fc0-483c-82f9-6ee33f65ebd9\"},{\"content\":{\"connectorIds\":[\"Out1\"],\"side\":\"RIGHT\"},\"type\":\"ConnectorPlacement.EquallySpacedRectSide\",\"uuid\":\"e11e5831-ab5e-42bb-bd0b-63825273f403\"},{\"content\":{\"connectorIds\":[\"In3\"],\"side\":\"TOP\"},\"type\":\"ConnectorPlacement.EquallySpacedRectSide\",\"uuid\":\"2b39bd07-2b6e-4e89-bb54-1321cea2c793\"},{\"content\":{\"connectorIds\":[],\"side\":\"HIDDEN\"},\"type\":\"ConnectorPlacement.EquallySpacedRectSide\",\"uuid\":\"a99c5943-5af0-4d11-8875-695bd24f17f4\"}]},\"type\":\"ConnectorPlacement.EquallySpacedConnector\",\"uuid\":\"a2a714db-f067-4e0e-8919-f68d1dab84ba\"}],\"packageUris\":[\"http://schema.mathworks.com/mf0/Connector/R2020b\"],\"version\":\"1.0\"}"
  Entkopplungszelle32 : Subsystem
      settings: PortSchema="{\"entries\":[{\"content\":{\"sides\":[{\"content\":{\"connectorIds\":[\"In1\",\"In2\"]},\"type\":\"ConnectorPlacement.EquallySpacedRectSide\",\"uuid\":\"e8e24803-2fc0-483c-82f9-6ee33f65ebd9\"},{\"content\":{\"connectorIds\":[\"Out1\"],\"side\":\"RIGHT\"},\"type\":\"ConnectorPlacement.EquallySpacedRectSide\",\"uuid\":\"e11e5831-ab5e-42bb-bd0b-63825273f403\"},{\"content\":{\"connectorIds\":[\"In3\"],\"side\":\"TOP\"},\"type\":\"ConnectorPlacement.EquallySpacedRectSide\",\"uuid\":\"2b39bd07-2b6e-4e89-bb54-1321cea2c793\"},{\"content\":{\"connectorIds\":[],\"side\":\"HIDDEN\"},\"type\":\"ConnectorPlacement.EquallySpacedRectSide\",\"uuid\":\"a99c5943-5af0-4d11-8875-695bd24f17f4\"}]},\"type\":\"ConnectorPlacement.EquallySpacedConnector\",\"uuid\":\"a2a714db-f067-4e0e-8919-f68d1dab84ba\"}],\"packageUris\":[\"http://schema.mathworks.com/mf0/Connector/R2020b\"],\"version\":\"1.0\"}"
  Entkopplungszelle33 : Subsystem
      settings: PortSchema="{\"entries\":[{\"content\":{\"sides\":[{\"content\":{\"connectorIds\":[\"In1\",\"In2\"]},\"type\":\"ConnectorPlacement.EquallySpacedRectSide\",\"uuid\":\"e8e24803-2fc0-483c-82f9-6ee33f65ebd9\"},{\"content\":{\"connectorIds\":[\"Out1\"],\"side\":\"RIGHT\"},\"type\":\"ConnectorPlacement.EquallySpacedRectSide\",\"uuid\":\"e11e5831-ab5e-42bb-bd0b-63825273f403\"},{\"content\":{\"connectorIds\":[\"In3\"],\"side\":\"TOP\"},\"type\":\"ConnectorPlacement.EquallySpacedRectSide\",\"uuid\":\"2b39bd07-2b6e-4e89-bb54-1321cea2c793\"},{\"content\":{\"connectorIds\":[],\"side\":\"HIDDEN\"},\"type\":\"ConnectorPlacement.EquallySpacedRectSide\",\"uuid\":\"a99c5943-5af0-4d11-8875-695bd24f17f4\"}]},\"type\":\"ConnectorPlacement.EquallySpacedConnector\",\"uuid\":\"a2a714db-f067-4e0e-8919-f68d1dab84ba\"}],\"packageUris\":[\"http://schema.mathworks.com/mf0/Connector/R2020b\"],\"version\":\"1.0\"}"
  Entkopplungszelle34 : Subsystem
      settings: PortSchema="{\"entries\":[{\"content\":{\"sides\":[{\"content\":{\"connectorIds\":[\"In1\",\"In2\"]},\"type\":\"ConnectorPlacement.EquallySpacedRectSide\",\"uuid\":\"e8e24803-2fc0-483c-82f9-6ee33f65ebd9\"},{\"content\":{\"connectorIds\":[\"Out1\"],\"side\":\"RIGHT\"},\"type\":\"ConnectorPlacement.EquallySpacedRectSide\",\"uuid\":\"e11e5831-ab5e-42bb-bd0b-63825273f403\"},{\"content\":{\"connectorIds\":[\"In3\"],\"side\":\"TOP\"},\"type\":\"ConnectorPlacement.EquallySpacedRectSide\",\"uuid\":\"2b39bd07-2b6e-4e89-bb54-1321cea2c793\"},{\"content\":{\"connectorIds\":[],\"side\":\"HIDDEN\"},\"type\":\"ConnectorPlacement.EquallySpacedRectSide\",\"uuid\":\"a99c5943-5af0-4d11-8875-695bd24f17f4\"}]},\"type\":\"ConnectorPlacement.EquallySpacedConnector\",\"uuid\":\"a2a714db-f067-4e0e-8919-f68d1dab84ba\"}],\"packageUris\":[\"http://schema.mathworks.com/mf0/Connector/R2020b\"],\"version\":\"1.0\"}"
  Entkopplungszelle35 : Subsystem
      settings: PortSchema="{\"entries\":[{\"content\":{\"sides\":[{\"content\":{\"connectorIds\":[\"In1\",\"In2\"]},\"type\":\"ConnectorPlacement.EquallySpacedRectSide\",\"uuid\":\"e8e24803-2fc0-483c-82f9-6ee33f65ebd9\"},{\"content\":{\"connectorIds\":[\"Out1\"],\"side\":\"RIGHT\"},\"type\":\"ConnectorPlacement.EquallySpacedRectSide\",\"uuid\":\"e11e5831-ab5e-42bb-bd0b-63825273f403\"},{\"content\":{\"connectorIds\":[\"In3\"],\"side\":\"TOP\"},\"type\":\"ConnectorPlacement.EquallySpacedRectSide\",\"uuid\":\"2b39bd07-2b6e-4e89-bb54-1321cea2c793\"},{\"content\":{\"connectorIds\":[],\"side\":\"HIDDEN\"},\"type\":\"ConnectorPlacement.EquallySpacedRectSide\",\"uuid\":\"a99c5943-5af0-4d11-8875-695bd24f17f4\"}]},\"type\":\"ConnectorPlacement.EquallySpacedConnector\",\"uuid\":\"a2a714db-f067-4e0e-8919-f68d1dab84ba\"}],\"packageUris\":[\"http://schema.mathworks.com/mf0/Connector/R2020b\"],\"version\":\"1.0\"}"
  Entkopplungszelle36 : Subsystem
      settings: PortSchema="{\"entries\":[{\"content\":{\"sides\":[{\"content\":{\"connectorIds\":[\"In1\",\"In2\"]},\"type\":\"ConnectorPlacement.EquallySpacedRectSide\",\"uuid\":\"e8e24803-2fc0-483c-82f9-6ee33f65ebd9\"},{\"content\":{\"connectorIds\":[\"Out1\"],\"side\":\"RIGHT\"},\"type\":\"ConnectorPlacement.EquallySpacedRectSide\",\"uuid\":\"e11e5831-ab5e-42bb-bd0b-63825273f403\"},{\"content\":{\"connectorIds\":[\"In3\"],\"side\":\"TOP\"},\"type\":\"ConnectorPlacement.EquallySpacedRectSide\",\"uuid\":\"2b39bd07-2b6e-4e89-bb54-1321cea2c793\"},{\"content\":{\"connectorIds\":[],\"side\":\"HIDDEN\"},\"type\":\"ConnectorPlacement.EquallySpacedRectSide\",\"uuid\":\"a99c5943-5af0-4d11-8875-695bd24f17f4\"}]},\"type\":\"ConnectorPlacement.EquallySpacedConnector\",\"uuid\":\"a2a714db-f067-4e0e-8919-f68d1dab84ba\"}],\"packageUris\":[\"http://schema.mathworks.com/mf0/Connector/R2020b\"],\"version\":\"1.0\"}"
  Entkopplungszelle37 : Subsystem
      settings: PortSchema="{\"entries\":[{\"content\":{\"sides\":[{\"content\":{\"connectorIds\":[\"In1\",\"In2\"]},\"type\":\"ConnectorPlacement.EquallySpacedRectSide\",\"uuid\":\"e8e24803-2fc0-483c-82f9-6ee33f65ebd9\"},{\"content\":{\"connectorIds\":[\"Out1\"],\"side\":\"RIGHT\"},\"type\":\"ConnectorPlacement.EquallySpacedRectSide\",\"uuid\":\"e11e5831-ab5e-42bb-bd0b-63825273f403\"},{\"content\":{\"connectorIds\":[\"In3\"],\"side\":\"TOP\"},\"type\":\"ConnectorPlacement.EquallySpacedRectSide\",\"uuid\":\"2b39bd07-2b6e-4e89-bb54-1321cea2c793\"},{\"content\":{\"connectorIds\":[],\"side\":\"HIDDEN\"},\"type\":\"ConnectorPlacement.EquallySpacedRectSide\",\"uuid\":\"a99c5943-5af0-4d11-8875-695bd24f17f4\"}]},\"type\":\"ConnectorPlacement.EquallySpacedConnector\",\"uuid\":\"a2a714db-f067-4e0e-8919-f68d1dab84ba\"}],\"packageUris\":[\"http://schema.mathworks.com/mf0/Connector/R2020b\"],\"version\":\"1.0\"}"
  Entkopplungszelle38 : Subsystem
      settings: PortSchema="{\"entries\":[{\"content\":{\"sides\":[{\"content\":{\"connectorIds\":[\"In1\",\"In2\"]},\"type\":\"ConnectorPlacement.EquallySpacedRectSide\",\"uuid\":\"e8e24803-2fc0-483c-82f9-6ee33f65ebd9\"},{\"content\":{\"connectorIds\":[\"Out1\"],\"side\":\"RIGHT\"},\"type\":\"ConnectorPlacement.EquallySpacedRectSide\",\"uuid\":\"e11e5831-ab5e-42bb-bd0b-63825273f403\"},{\"content\":{\"connectorIds\":[\"In3\"],\"side\":\"TOP\"},\"type\":\"ConnectorPlacement.EquallySpacedRectSide\",\"uuid\":\"2b39bd07-2b6e-4e89-bb54-1321cea2c793\"},{\"content\":{\"connectorIds\":[],\"side\":\"HIDDEN\"},\"type\":\"ConnectorPlacement.EquallySpacedRectSide\",\"uuid\":\"a99c5943-5af0-4d11-8875-695bd24f17f4\"}]},\"type\":\"ConnectorPlacement.EquallySpacedConnector\",\"uuid\":\"a2a714db-f067-4e0e-8919-f68d1dab84ba\"}],\"packageUris\":[\"http://schema.mathworks.com/mf0/Connector/R2020b\"],\"version\":\"1.0\"}"
  Entkopplungszelle39 : Subsystem
      settings: PortSchema="{\"entries\":[{\"content\":{\"sides\":[{\"content\":{\"connectorIds\":[\"In1\",\"In2\"]},\"type\":\"ConnectorPlacement.EquallySpacedRectSide\",\"uuid\":\"e8e24803-2fc0-483c-82f9-6ee33f65ebd9\"},{\"content\":{\"connectorIds\":[\"Out1\"],\"side\":\"RIGHT\"},\"type\":\"ConnectorPlacement.EquallySpacedRectSide\",\"uuid\":\"e11e5831-ab5e-42bb-bd0b-63825273f403\"},{\"content\":{\"connectorIds\":[\"In3\"],\"side\":\"TOP\"},\"type\":\"ConnectorPlacement.EquallySpacedRectSide\",\"uuid\":\"2b39bd07-2b6e-4e89-bb54-1321cea2c793\"},{\"content\":{\"connectorIds\":[],\"side\":\"HIDDEN\"},\"type\":\"ConnectorPlacement.EquallySpacedRectSide\",\"uuid\":\"a99c5943-5af0-4d11-8875-695bd24f17f4\"}]},\"type\":\"ConnectorPlacement.EquallySpacedConnector\",\"uuid\":\"a2a714db-f067-4e0e-8919-f68d1dab84ba\"}],\"packageUris\":[\"http://schema.mathworks.com/mf0/Connector/R2020b\"],\"version\":\"1.0\"}"
  Entkopplungszelle4 : Subsystem
      settings: PortSchema="{\"entries\":[{\"content\":{\"sides\":[{\"content\":{\"connectorIds\":[\"In1\",\"In2\"]},\"type\":\"ConnectorPlacement.EquallySpacedRectSide\",\"uuid\":\"e8e24803-2fc0-483c-82f9-6ee33f65ebd9\"},{\"content\":{\"connectorIds\":[\"Out1\"],\"side\":\"RIGHT\"},\"type\":\"ConnectorPlacement.EquallySpacedRectSide\",\"uuid\":\"e11e5831-ab5e-42bb-bd0b-63825273f403\"},{\"content\":{\"connectorIds\":[\"In3\"],\"side\":\"TOP\"},\"type\":\"ConnectorPlacement.EquallySpacedRectSide\",\"uuid\":\"2b39bd07-2b6e-4e89-bb54-1321cea2c793\"},{\"content\":{\"connectorIds\":[],\"side\":\"HIDDEN\"},\"type\":\"ConnectorPlacement.EquallySpacedRectSide\",\"uuid\":\"a99c5943-5af0-4d11-8875-695bd24f17f4\"}]},\"type\":\"ConnectorPlacement.EquallySpacedConnector\",\"uuid\":\"a2a714db-f067-4e0e-8919-f68d1dab84ba\"}],\"packageUris\":[\"http://schema.mathworks.com/mf0/Connector/R2020b\"],\"version\":\"1.0\"}"
  Entkopplungszelle40 : Subsystem
      settings: PortSchema="{\"entries\":[{\"content\":{\"sides\":[{\"content\":{\"connectorIds\":[\"In1\",\"In2\"]},\"type\":\"ConnectorPlacement.EquallySpacedRectSide\",\"uuid\":\"e8e24803-2fc0-483c-82f9-6ee33f65ebd9\"},{\"content\":{\"connectorIds\":[\"Out1\"],\"side\":\"RIGHT\"},\"type\":\"ConnectorPlacement.EquallySpacedRectSide\",\"uuid\":\"e11e5831-ab5e-42bb-bd0b-63825273f403\"},{\"content\":{\"connectorIds\":[\"In3\"],\"side\":\"TOP\"},\"type\":\"ConnectorPlacement.EquallySpacedRectSide\",\"uuid\":\"2b39bd07-2b6e-4e89-bb54-1321cea2c793\"},{\"content\":{\"connectorIds\":[],\"side\":\"HIDDEN\"},\"type\":\"ConnectorPlacement.EquallySpacedRectSide\",\"uuid\":\"a99c5943-5af0-4d11-8875-695bd24f17f4\"}]},\"type\":\"ConnectorPlacement.EquallySpacedConnector\",\"uuid\":\"a2a714db-f067-4e0e-8919-f68d1dab84ba\"}],\"packageUris\":[\"http://schema.mathworks.com/mf0/Connector/R2020b\"],\"version\":\"1.0\"}"
  Entkopplungszelle41 : Subsystem
      settings: PortSchema="{\"entries\":[{\"content\":{\"sides\":[{\"content\":{\"connectorIds\":[\"In1\",\"In2\"]},\"type\":\"ConnectorPlacement.EquallySpacedRectSide\",\"uuid\":\"e8e24803-2fc0-483c-82f9-6ee33f65ebd9\"},{\"content\":{\"connectorIds\":[\"Out1\"],\"side\":\"RIGHT\"},\"type\":\"ConnectorPlacement.EquallySpacedRectSide\",\"uuid\":\"e11e5831-ab5e-42bb-bd0b-63825273f403\"},{\"content\":{\"connectorIds\":[\"In3\"],\"side\":\"TOP\"},\"type\":\"ConnectorPlacement.EquallySpacedRectSide\",\"uuid\":\"2b39bd07-2b6e-4e89-bb54-1321cea2c793\"},{\"content\":{\"connectorIds\":[],\"side\":\"HIDDEN\"},\"type\":\"ConnectorPlacement.EquallySpacedRectSide\",\"uuid\":\"a99c5943-5af0-4d11-8875-695bd24f17f4\"}]},\"type\":\"ConnectorPlacement.EquallySpacedConnector\",\"uuid\":\"a2a714db-f067-4e0e-8919-f68d1dab84ba\"}],\"packageUris\":[\"http://schema.mathworks.com/mf0/Connector/R2020b\"],\"version\":\"1.0\"}"
  Entkopplungszelle42 : Subsystem
      settings: PortSchema="{\"entries\":[{\"content\":{\"sides\":[{\"content\":{\"connectorIds\":[\"In1\",\"In2\"]},\"type\":\"ConnectorPlacement.EquallySpacedRectSide\",\"uuid\":\"e8e24803-2fc0-483c-82f9-6ee33f65ebd9\"},{\"content\":{\"connectorIds\":[\"Out1\"],\"side\":\"RIGHT\"},\"type\":\"ConnectorPlacement.EquallySpacedRectSide\",\"uuid\":\"e11e5831-ab5e-42bb-bd0b-63825273f403\"},{\"content\":{\"connectorIds\":[\"In3\"],\"side\":\"TOP\"},\"type\":\"ConnectorPlacement.EquallySpacedRectSide\",\"uuid\":\"2b39bd07-2b6e-4e89-bb54-1321cea2c793\"},{\"content\":{\"connectorIds\":[],\"side\":\"HIDDEN\"},\"type\":\"ConnectorPlacement.EquallySpacedRectSide\",\"uuid\":\"a99c5943-5af0-4d11-8875-695bd24f17f4\"}]},\"type\":\"ConnectorPlacement.EquallySpacedConnector\",\"uuid\":\"a2a714db-f067-4e0e-8919-f68d1dab84ba\"}],\"packageUris\":[\"http://schema.mathworks.com/mf0/Connector/R2020b\"],\"version\":\"1.0\"}"
  Entkopplungszelle43 : Subsystem
      settings: PortSchema="{\"entries\":[{\"content\":{\"sides\":[{\"content\":{\"connectorIds\":[\"In1\",\"In2\"]},\"type\":\"ConnectorPlacement.EquallySpacedRectSide\",\"uuid\":\"e8e24803-2fc0-483c-82f9-6ee33f65ebd9\"},{\"content\":{\"connectorIds\":[\"Out1\"],\"side\":\"RIGHT\"},\"type\":\"ConnectorPlacement.EquallySpacedRectSide\",\"uuid\":\"e11e5831-ab5e-42bb-bd0b-63825273f403\"},{\"content\":{\"connectorIds\":[\"In3\"],\"side\":\"TOP\"},\"type\":\"ConnectorPlacement.EquallySpacedRectSide\",\"uuid\":\"2b39bd07-2b6e-4e89-bb54-1321cea2c793\"},{\"content\":{\"connectorIds\":[],\"side\":\"HIDDEN\"},\"type\":\"ConnectorPlacement.EquallySpacedRectSide\",\"uuid\":\"a99c5943-5af0-4d11-8875-695bd24f17f4\"}]},\"type\":\"ConnectorPlacement.EquallySpacedConnector\",\"uuid\":\"a2a714db-f067-4e0e-8919-f68d1dab84ba\"}],\"packageUris\":[\"http://schema.mathworks.com/mf0/Connector/R2020b\"],\"version\":\"1.0\"}"
  Entkopplungszelle44 : Subsystem
      settings: PortSchema="{\"entries\":[{\"content\":{\"sides\":[{\"content\":{\"connectorIds\":[\"In1\",\"In2\"]},\"type\":\"ConnectorPlacement.EquallySpacedRectSide\",\"uuid\":\"e8e24803-2fc0-483c-82f9-6ee33f65ebd9\"},{\"content\":{\"connectorIds\":[\"Out1\"],\"side\":\"RIGHT\"},\"type\":\"ConnectorPlacement.EquallySpacedRectSide\",\"uuid\":\"e11e5831-ab5e-42bb-bd0b-63825273f403\"},{\"content\":{\"connectorIds\":[\"In3\"],\"side\":\"TOP\"},\"type\":\"ConnectorPlacement.EquallySpacedRectSide\",\"uuid\":\"2b39bd07-2b6e-4e89-bb54-1321cea2c793\"},{\"content\":{\"connectorIds\":[],\"side\":\"HIDDEN\"},\"type\":\"ConnectorPlacement.EquallySpacedRectSide\",\"uuid\":\"a99c5943-5af0-4d11-8875-695bd24f17f4\"}]},\"type\":\"ConnectorPlacement.EquallySpacedConnector\",\"uuid\":\"a2a714db-f067-4e0e-8919-f68d1dab84ba\"}],\"packageUris\":[\"http://schema.mathworks.com/mf0/Connector/R2020b\"],\"version\":\"1.0\"}"
  Entkopplungszelle45 : Subsystem
      settings: PortSchema="{\"entries\":[{\"content\":{\"sides\":[{\"content\":{\"connectorIds\":[\"In1\",\"In2\"]},\"type\":\"ConnectorPlacement.EquallySpacedRectSide\",\"uuid\":\"e8e24803-2fc0-483c-82f9-6ee33f65ebd9\"},{\"content\":{\"connectorIds\":[\"Out1\"],\"side\":\"RIGHT\"},\"type\":\"ConnectorPlacement.EquallySpacedRectSide\",\"uuid\":\"e11e5831-ab5e-42bb-bd0b-63825273f403\"},{\"content\":{\"connectorIds\":[\"In3\"],\"side\":\"TOP\"},\"type\":\"ConnectorPlacement.EquallySpacedRectSide\",\"uuid\":\"2b39bd07-2b6e-4e89-bb54-1321cea2c793\"},{\"content\":{\"connectorIds\":[],\"side\":\"HIDDEN\"},\"type\":\"ConnectorPlacement.EquallySpacedRectSide\",\"uuid\":\"a99c5943-5af0-4d11-8875-695bd24f17f4\"}]},\"type\":\"ConnectorPlacement.EquallySpacedConnector\",\"uuid\":\"a2a714db-f067-4e0e-8919-f68d1dab84ba\"}],\"packageUris\":[\"http://schema.mathworks.com/mf0/Connector/R2020b\"],\"version\":\"1.0\"}"
  Entkopplungszelle46 : Subsystem
      settings: PortSchema="{\"entries\":[{\"content\":{\"sides\":[{\"content\":{\"connectorIds\":[\"In1\",\"In2\"]},\"type\":\"ConnectorPlacement.EquallySpacedRectSide\",\"uuid\":\"e8e24803-2fc0-483c-82f9-6ee33f65ebd9\"},{\"content\":{\"connectorIds\":[\"Out1\"],\"side\":\"RIGHT\"},\"type\":\"ConnectorPlacement.EquallySpacedRectSide\",\"uuid\":\"e11e5831-ab5e-42bb-bd0b-63825273f403\"},{\"content\":{\"connectorIds\":[\"In3\"],\"side\":\"TOP\"},\"type\":\"ConnectorPlacement.EquallySpacedRectSide\",\"uuid\":\"2b39bd07-2b6e-4e89-bb54-1321cea2c793\"},{\"content\":{\"connectorIds\":[],\"side\":\"HIDDEN\"},\"type\":\"ConnectorPlacement.EquallySpacedRectSide\",\"uuid\":\"a99c5943-5af0-4d11-8875-695bd24f17f4\"}]},\"type\":\"ConnectorPlacement.EquallySpacedConnector\",\"uuid\":\"a2a714db-f067-4e0e-8919-f68d1dab84ba\"}],\"packageUris\":[\"http://schema.mathworks.com/mf0/Connector/R2020b\"],\"version\":\"1.0\"}"
  Entkopplungszelle47 : Subsystem
      settings: PortSchema="{\"entries\":[{\"content\":{\"sides\":[{\"content\":{\"connectorIds\":[\"In1\",\"In2\"]},\"type\":\"ConnectorPlacement.EquallySpacedRectSide\",\"uuid\":\"e8e24803-2fc0-483c-82f9-6ee33f65ebd9\"},{\"content\":{\"connectorIds\":[\"Out1\"],\"side\":\"RIGHT\"},\"type\":\"ConnectorPlacement.EquallySpacedRectSide\",\"uuid\":\"e11e5831-ab5e-42bb-bd0b-63825273f403\"},{\"content\":{\"connectorIds\":[\"In3\"],\"side\":\"TOP\"},\"type\":\"ConnectorPlacement.EquallySpacedRectSide\",\"uuid\":\"2b39bd07-2b6e-4e89-bb54-1321cea2c793\"},{\"content\":{\"connectorIds\":[],\"side\":\"HIDDEN\"},\"type\":\"ConnectorPlacement.EquallySpacedRectSide\",\"uuid\":\"a99c5943-5af0-4d11-8875-695bd24f17f4\"}]},\"type\":\"ConnectorPlacement.EquallySpacedConnector\",\"uuid\":\"a2a714db-f067-4e0e-8919-f68d1dab84ba\"}],\"packageUris\":[\"http://schema.mathworks.com/mf0/Connector/R2020b\"],\"version\":\"1.0\"}"
  Entkopplungszelle48 : Subsystem
      settings: PortSchema="{\"entries\":[{\"content\":{\"sides\":[{\"content\":{\"connectorIds\":[\"In1\",\"In2\"]},\"type\":\"ConnectorPlacement.EquallySpacedRectSide\",\"uuid\":\"e8e24803-2fc0-483c-82f9-6ee33f65ebd9\"},{\"content\":{\"connectorIds\":[\"Out1\"],\"side\":\"RIGHT\"},\"type\":\"ConnectorPlacement.EquallySpacedRectSide\",\"uuid\":\"e11e5831-ab5e-42bb-bd0b-63825273f403\"},{\"content\":{\"connectorIds\":[\"In3\"],\"side\":\"TOP\"},\"type\":\"ConnectorPlacement.EquallySpacedRectSide\",\"uuid\":\"2b39bd07-2b6e-4e89-bb54-1321cea2c793\"},{\"content\":{\"connectorIds\":[],\"side\":\"HIDDEN\"},\"type\":\"ConnectorPlacement.EquallySpacedRectSide\",\"uuid\":\"a99c5943-5af0-4d11-8875-695bd24f17f4\"}]},\"type\":\"ConnectorPlacement.EquallySpacedConnector\",\"uuid\":\"a2a714db-f067-4e0e-8919-f68d1dab84ba\"}],\"packageUris\":[\"http://schema.mathworks.com/mf0/Connector/R2020b\"],\"version\":\"1.0\"}"
  Entkopplungszelle49 : Subsystem
      settings: PortSchema="{\"entries\":[{\"content\":{\"sides\":[{\"content\":{\"connectorIds\":[\"In1\",\"In2\"]},\"type\":\"ConnectorPlacement.EquallySpacedRectSide\",\"uuid\":\"e8e24803-2fc0-483c-82f9-6ee33f65ebd9\"},{\"content\":{\"connectorIds\":[\"Out1\"],\"side\":\"RIGHT\"},\"type\":\"ConnectorPlacement.EquallySpacedRectSide\",\"uuid\":\"e11e5831-ab5e-42bb-bd0b-63825273f403\"},{\"content\":{\"connectorIds\":[\"In3\"],\"side\":\"TOP\"},\"type\":\"ConnectorPlacement.EquallySpacedRectSide\",\"uuid\":\"2b39bd07-2b6e-4e89-bb54-1321cea2c793\"},{\"content\":{\"connectorIds\":[],\"side\":\"HIDDEN\"},\"type\":\"ConnectorPlacement.EquallySpacedRectSide\",\"uuid\":\"a99c5943-5af0-4d11-8875-695bd24f17f4\"}]},\"type\":\"ConnectorPlacement.EquallySpacedConnector\",\"uuid\":\"a2a714db-f067-4e0e-8919-f68d1dab84ba\"}],\"packageUris\":[\"http://schema.mathworks.com/mf0/Connector/R2020b\"],\"version\":\"1.0\"}"
  Entkopplungszelle5 : Subsystem
      settings: PortSchema="{\"entries\":[{\"content\":{\"sides\":[{\"content\":{\"connectorIds\":[\"In1\",\"In2\"]},\"type\":\"ConnectorPlacement.EquallySpacedRectSide\",\"uuid\":\"e8e24803-2fc0-483c-82f9-6ee33f65ebd9\"},{\"content\":{\"connectorIds\":[\"Out1\"],\"side\":\"RIGHT\"},\"type\":\"ConnectorPlacement.EquallySpacedRectSide\",\"uuid\":\"e11e5831-ab5e-42bb-bd0b-63825273f403\"},{\"content\":{\"connectorIds\":[\"In3\"],\"side\":\"TOP\"},\"type\":\"ConnectorPlacement.EquallySpacedRectSide\",\"uuid\":\"2b39bd07-2b6e-4e89-bb54-1321cea2c793\"},{\"content\":{\"connectorIds\":[],\"side\":\"HIDDEN\"},\"type\":\"ConnectorPlacement.EquallySpacedRectSide\",\"uuid\":\"a99c5943-5af0-4d11-8875-695bd24f17f4\"}]},\"type\":\"ConnectorPlacement.EquallySpacedConnector\",\"uuid\":\"a2a714db-f067-4e0e-8919-f68d1dab84ba\"}],\"packageUris\":[\"http://schema.mathworks.com/mf0/Connector/R2020b\"],\"version\":\"1.0\"}"
  Entkopplungszelle50 : Subsystem
      settings: PortSchema="{\"entries\":[{\"content\":{\"sides\":[{\"content\":{\"connectorIds\":[\"In1\",\"In2\"]},\"type\":\"ConnectorPlacement.EquallySpacedRectSide\",\"uuid\":\"e8e24803-2fc0-483c-82f9-6ee33f65ebd9\"},{\"content\":{\"connectorIds\":[\"Out1\"],\"side\":\"RIGHT\"},\"type\":\"ConnectorPlacement.EquallySpacedRectSide\",\"uuid\":\"e11e5831-ab5e-42bb-bd0b-63825273f403\"},{\"content\":{\"connectorIds\":[\"In3\"],\"side\":\"TOP\"},\"type\":\"ConnectorPlacement.EquallySpacedRectSide\",\"uuid\":\"2b39bd07-2b6e-4e89-bb54-1321cea2c793\"},{\"content\":{\"connectorIds\":[],\"side\":\"HIDDEN\"},\"type\":\"ConnectorPlacement.EquallySpacedRectSide\",\"uuid\":\"a99c5943-5af0-4d11-8875-695bd24f17f4\"}]},\"type\":\"ConnectorPlacement.EquallySpacedConnector\",\"uuid\":\"a2a714db-f067-4e0e-8919-f68d1dab84ba\"}],\"packageUris\":[\"http://schema.mathworks.com/mf0/Connector/R2020b\"],\"version\":\"1.0\"}"
  Entkopplungszelle51 : Subsystem
      settings: PortSchema="{\"entries\":[{\"content\":{\"sides\":[{\"content\":{\"connectorIds\":[\"In1\",\"In2\"]},\"type\":\"ConnectorPlacement.EquallySpacedRectSide\",\"uuid\":\"e8e24803-2fc0-483c-82f9-6ee33f65ebd9\"},{\"content\":{\"connectorIds\":[\"Out1\"],\"side\":\"RIGHT\"},\"type\":\"ConnectorPlacement.EquallySpacedRectSide\",\"uuid\":\"e11e5831-ab5e-42bb-bd0b-63825273f403\"},{\"content\":{\"connectorIds\":[\"In3\"],\"side\":\"TOP\"},\"type\":\"ConnectorPlacement.EquallySpacedRectSide\",\"uuid\":\"2b39bd07-2b6e-4e89-bb54-1321cea2c793\"},{\"content\":{\"connectorIds\":[],\"side\":\"HIDDEN\"},\"type\":\"ConnectorPlacement.EquallySpacedRectSide\",\"uuid\":\"a99c5943-5af0-4d11-8875-695bd24f17f4\"}]},\"type\":\"ConnectorPlacement.EquallySpacedConnector\",\"uuid\":\"a2a714db-f067-4e0e-8919-f68d1dab84ba\"}],\"packageUris\":[\"http://schema.mathworks.com/mf0/Connector/R2020b\"],\"version\":\"1.0\"}"
  Entkopplungszelle52 : Subsystem
      settings: PortSchema="{\"entries\":[{\"content\":{\"sides\":[{\"content\":{\"connectorIds\":[\"In1\",\"In2\"]},\"type\":\"ConnectorPlacement.EquallySpacedRectSide\",\"uuid\":\"e8e24803-2fc0-483c-82f9-6ee33f65ebd9\"},{\"content\":{\"connectorIds\":[\"Out1\"],\"side\":\"RIGHT\"},\"type\":\"ConnectorPlacement.EquallySpacedRectSide\",\"uuid\":\"e11e5831-ab5e-42bb-bd0b-63825273f403\"},{\"content\":{\"connectorIds\":[\"In3\"],\"side\":\"TOP\"},\"type\":\"ConnectorPlacement.EquallySpacedRectSide\",\"uuid\":\"2b39bd07-2b6e-4e89-bb54-1321cea2c793\"},{\"content\":{\"connectorIds\":[],\"side\":\"HIDDEN\"},\"type\":\"ConnectorPlacement.EquallySpacedRectSide\",\"uuid\":\"a99c5943-5af0-4d11-8875-695bd24f17f4\"}]},\"type\":\"ConnectorPlacement.EquallySpacedConnector\",\"uuid\":\"a2a714db-f067-4e0e-8919-f68d1dab84ba\"}],\"packageUris\":[\"http://schema.mathworks.com/mf0/Connector/R2020b\"],\"version\":\"1.0\"}"
  Entkopplungszelle53 : Subsystem
      settings: PortSchema="{\"entries\":[{\"content\":{\"sides\":[{\"content\":{\"connectorIds\":[\"In1\",\"In2\"]},\"type\":\"ConnectorPlacement.EquallySpacedRectSide\",\"uuid\":\"e8e24803-2fc0-483c-82f9-6ee33f65ebd9\"},{\"content\":{\"connectorIds\":[\"Out1\"],\"side\":\"RIGHT\"},\"type\":\"ConnectorPlacement.EquallySpacedRectSide\",\"uuid\":\"e11e5831-ab5e-42bb-bd0b-63825273f403\"},{\"content\":{\"connectorIds\":[\"In3\"],\"side\":\"TOP\"},\"type\":\"ConnectorPlacement.EquallySpacedRectSide\",\"uuid\":\"2b39bd07-2b6e-4e89-bb54-1321cea2c793\"},{\"content\":{\"connectorIds\":[],\"side\":\"HIDDEN\"},\"type\":\"ConnectorPlacement.EquallySpacedRectSide\",\"uuid\":\"a99c5943-5af0-4d11-8875-695bd24f17f4\"}]},\"type\":\"ConnectorPlacement.EquallySpacedConnector\",\"uuid\":\"a2a714db-f067-4e0e-8919-f68d1dab84ba\"}],\"packageUris\":[\"http://schema.mathworks.com/mf0/Connector/R2020b\"],\"version\":\"1.0\"}"
  Entkopplungszelle54 : Subsystem
      settings: PortSchema="{\"entries\":[{\"content\":{\"sides\":[{\"content\":{\"connectorIds\":[\"In1\",\"In2\"]},\"type\":\"ConnectorPlacement.EquallySpacedRectSide\",\"uuid\":\"e8e24803-2fc0-483c-82f9-6ee33f65ebd9\"},{\"content\":{\"connectorIds\":[\"Out1\"],\"side\":\"RIGHT\"},\"type\":\"ConnectorPlacement.EquallySpacedRectSide\",\"uuid\":\"e11e5831-ab5e-42bb-bd0b-63825273f403\"},{\"content\":{\"connectorIds\":[\"In3\"],\"side\":\"TOP\"},\"type\":\"ConnectorPlacement.EquallySpacedRectSide\",\"uuid\":\"2b39bd07-2b6e-4e89-bb54-1321cea2c793\"},{\"content\":{\"connectorIds\":[],\"side\":\"HIDDEN\"},\"type\":\"ConnectorPlacement.EquallySpacedRectSide\",\"uuid\":\"a99c5943-5af0-4d11-8875-695bd24f17f4\"}]},\"type\":\"ConnectorPlacement.EquallySpacedConnector\",\"uuid\":\"a2a714db-f067-4e0e-8919-f68d1dab84ba\"}],\"packageUris\":[\"http://schema.mathworks.com/mf0/Connector/R2020b\"],\"version\":\"1.0\"}"
  Entkopplungszelle55 : Subsystem
      settings: PortSchema="{\"entries\":[{\"content\":{\"sides\":[{\"content\":{\"connectorIds\":[\"In1\",\"In2\"]},\"type\":\"ConnectorPlacement.EquallySpacedRectSide\",\"uuid\":\"e8e24803-2fc0-483c-82f9-6ee33f65ebd9\"},{\"content\":{\"connectorIds\":[\"Out1\"],\"side\":\"RIGHT\"},\"type\":\"ConnectorPlacement.EquallySpacedRectSide\",\"uuid\":\"e11e5831-ab5e-42bb-bd0b-63825273f403\"},{\"content\":{\"connectorIds\":[\"In3\"],\"side\":\"TOP\"},\"type\":\"ConnectorPlacement.EquallySpacedRectSide\",\"uuid\":\"2b39bd07-2b6e-4e89-bb54-1321cea2c793\"},{\"content\":{\"connectorIds\":[],\"side\":\"HIDDEN\"},\"type\":\"ConnectorPlacement.EquallySpacedRectSide\",\"uuid\":\"a99c5943-5af0-4d11-8875-695bd24f17f4\"}]},\"type\":\"ConnectorPlacement.EquallySpacedConnector\",\"uuid\":\"a2a714db-f067-4e0e-8919-f68d1dab84ba\"}],\"packageUris\":[\"http://schema.mathworks.com/mf0/Connector/R2020b\"],\"version\":\"1.0\"}"
  Entkopplungszelle56 : Subsystem
      settings: PortSchema="{\"entries\":[{\"content\":{\"sides\":[{\"content\":{\"connectorIds\":[\"In1\",\"In2\"]},\"type\":\"ConnectorPlacement.EquallySpacedRectSide\",\"uuid\":\"e8e24803-2fc0-483c-82f9-6ee33f65ebd9\"},{\"content\":{\"connectorIds\":[\"Out1\"],\"side\":\"RIGHT\"},\"type\":\"ConnectorPlacement.EquallySpacedRectSide\",\"uuid\":\"e11e5831-ab5e-42bb-bd0b-63825273f403\"},{\"content\":{\"connectorIds\":[\"In3\"],\"side\":\"TOP\"},\"type\":\"ConnectorPlacement.EquallySpacedRectSide\",\"uuid\":\"2b39bd07-2b6e-4e89-bb54-1321cea2c793\"},{\"content\":{\"connectorIds\":[],\"side\":\"HIDDEN\"},\"type\":\"ConnectorPlacement.EquallySpacedRectSide\",\"uuid\":\"a99c5943-5af0-4d11-8875-695bd24f17f4\"}]},\"type\":\"ConnectorPlacement.EquallySpacedConnector\",\"uuid\":\"a2a714db-f067-4e0e-8919-f68d1dab84ba\"}],\"packageUris\":[\"http://schema.mathworks.com/mf0/Connector/R2020b\"],\"version\":\"1.0\"}"
  Entkopplungszelle6 : Subsystem
      settings: PortSchema="{\"entries\":[{\"content\":{\"sides\":[{\"content\":{\"connectorIds\":[\"In1\",\"In2\"]},\"type\":\"ConnectorPlacement.EquallySpacedRectSide\",\"uuid\":\"e8e24803-2fc0-483c-82f9-6ee33f65ebd9\"},{\"content\":{\"connectorIds\":[\"Out1\"],\"side\":\"RIGHT\"},\"type\":\"ConnectorPlacement.EquallySpacedRectSide\",\"uuid\":\"e11e5831-ab5e-42bb-bd0b-63825273f403\"},{\"content\":{\"connectorIds\":[\"In3\"],\"side\":\"TOP\"},\"type\":\"ConnectorPlacement.EquallySpacedRectSide\",\"uuid\":\"2b39bd07-2b6e-4e89-bb54-1321cea2c793\"},{\"content\":{\"connectorIds\":[],\"side\":\"HIDDEN\"},\"type\":\"ConnectorPlacement.EquallySpacedRectSide\",\"uuid\":\"a99c5943-5af0-4d11-8875-695bd24f17f4\"}]},\"type\":\"ConnectorPlacement.EquallySpacedConnector\",\"uuid\":\"a2a714db-f067-4e0e-8919-f68d1dab84ba\"}],\"packageUris\":[\"http://schema.mathworks.com/mf0/Connector/R2020b\"],\"version\":\"1.0\"}"
  Entkopplungszelle7 : Subsystem
      settings: PortSchema="{\"entries\":[{\"content\":{\"sides\":[{\"content\":{\"connectorIds\":[\"In1\",\"In2\"]},\"type\":\"ConnectorPlacement.EquallySpacedRectSide\",\"uuid\":\"e8e24803-2fc0-483c-82f9-6ee33f65ebd9\"},{\"content\":{\"connectorIds\":[\"Out1\"],\"side\":\"RIGHT\"},\"type\":\"ConnectorPlacement.EquallySpacedRectSide\",\"uuid\":\"e11e5831-ab5e-42bb-bd0b-63825273f403\"},{\"content\":{\"connectorIds\":[\"In3\"],\"side\":\"TOP\"},\"type\":\"ConnectorPlacement.EquallySpacedRectSide\",\"uuid\":\"2b39bd07-2b6e-4e89-bb54-1321cea2c793\"},{\"content\":{\"connectorIds\":[],\"side\":\"HIDDEN\"},\"type\":\"ConnectorPlacement.EquallySpacedRectSide\",\"uuid\":\"a99c5943-5af0-4d11-8875-695bd24f17f4\"}]},\"type\":\"ConnectorPlacement.EquallySpacedConnector\",\"uuid\":\"a2a714db-f067-4e0e-8919-f68d1dab84ba\"}],\"packageUris\":[\"http://schema.mathworks.com/mf0/Connector/R2020b\"],\"version\":\"1.0\"}"
  Entkopplungszelle8 : Subsystem
      settings: PortSchema="{\"entries\":[{\"content\":{\"sides\":[{\"content\":{\"connectorIds\":[\"In1\",\"In2\"]},\"type\":\"ConnectorPlacement.EquallySpacedRectSide\",\"uuid\":\"e8e24803-2fc0-483c-82f9-6ee33f65ebd9\"},{\"content\":{\"connectorIds\":[\"Out1\"],\"side\":\"RIGHT\"},\"type\":\"ConnectorPlacement.EquallySpacedRectSide\",\"uuid\":\"e11e5831-ab5e-42bb-bd0b-63825273f403\"},{\"content\":{\"connectorIds\":[\"In3\"],\"side\":\"TOP\"},\"type\":\"ConnectorPlacement.EquallySpacedRectSide\",\"uuid\":\"2b39bd07-2b6e-4e89-bb54-1321cea2c793\"},{\"content\":{\"connectorIds\":[],\"side\":\"HIDDEN\"},\"type\":\"ConnectorPlacement.EquallySpacedRectSide\",\"uuid\":\"a99c5943-5af0-4d11-8875-695bd24f17f4\"}]},\"type\":\"ConnectorPlacement.EquallySpacedConnector\",\"uuid\":\"a2a714db-f067-4e0e-8919-f68d1dab84ba\"}],\"packageUris\":[\"http://schema.mathworks.com/mf0/Connector/R2020b\"],\"version\":\"1.0\"}"
  Entkopplungszelle9 : Subsystem
      settings: PortSchema="{\"entries\":[{\"content\":{\"sides\":[{\"content\":{\"connectorIds\":[\"In1\",\"In2\"]},\"type\":\"ConnectorPlacement.EquallySpacedRectSide\",\"uuid\":\"e8e24803-2fc0-483c-82f9-6ee33f65ebd9\"},{\"content\":{\"connectorIds\":[\"Out1\"],\"side\":\"RIGHT\"},\"type\":\"ConnectorPlacement.EquallySpacedRectSide\",\"uuid\":\"e11e5831-ab5e-42bb-bd0b-63825273f403\"},{\"content\":{\"connectorIds\":[\"In3\"],\"side\":\"TOP\"},\"type\":\"ConnectorPlacement.EquallySpacedRectSide\",\"uuid\":\"2b39bd07-2b6e-4e89-bb54-1321cea2c793\"},{\"content\":{\"connectorIds\":[],\"side\":\"HIDDEN\"},\"type\":\"ConnectorPlacement.EquallySpacedRectSide\",\"uuid\":\"a99c5943-5af0-4d11-8875-695bd24f17f4\"}]},\"type\":\"ConnectorPlacement.EquallySpacedConnector\",\"uuid\":\"a2a714db-f067-4e0e-8919-f68d1dab84ba\"}],\"packageUris\":[\"http://schema.mathworks.com/mf0/Connector/R2020b\"],\"version\":\"1.0\"}"
  First-Order Filter{1..8} (8 alike) : powerlib_meascontrol/Filters/First-Order Filter  FilterType=Lowpass  Tc=1/(2*pi*5/sqrt(2))  Ts=0  Initialize=off  Vac_Init=[0, 0, 60]  Vdc_Init=0  PlotResponse=off  FreqRange="[0,  30,  1]"
  Gain{,16..19,33,68..71} (10 alike) : Gain
  Gain1 : Gain  Gain=2
  Gain10 : Gain  Gain=5
  Gain11 : Gain  Gain=9
  Gain12 : Gain  Gain=-5
  Gain{13,37,39,48} (4 alike) : Gain  Gain=-6
  Gain14 : Gain  Gain=-4
  Gain15 : Gain  Gain=-9
  Gain{2,24,35,45,51} (5 alike) : Gain  Gain=-3
  Gain20 : Gain  Gain=-2
  Gain21 : Gain  Gain=7
  Gain22 : Gain  Gain=-8
  Gain23 : Gain  Gain=19
  Gain{3,25,34,59} (4 alike) : Gain  Gain=6
  Gain26 : Gain  Gain=-9
  Gain27 : Gain  Gain=18
  Gain28 : Gain  Gain=-1
  Gain29 : Gain  Gain=8
  Gain30 : Gain  Gain=-7
  Gain31 : Gain  Gain=20
  Gain{9,32,40..41,57} (5 alike) : Gain  Gain=3
  Gain36 : Gain  Gain=9
  Gain38 : Gain  Gain=21
  Gain4 : Gain  Gain=-1
  Gain42 : Gain  Gain=-12
  Gain43 : Gain  Gain=15
  Gain44 : Gain  Gain=12
  Gain46 : Gain  Gain=24
  Gain47 : Gain  Gain=-12
  Gain49 : Gain  Gain=-8
  Gain5 : Gain  Gain=-2
  Gain50 : Gain  Gain=-9
  Gain52 : Gain  Gain=15
  Gain53 : Gain  Gain=-15
  Gain54 : Gain  Gain=12
  Gain55 : Gain  Gain=-27
  Gain56 : Gain  Gain=27
  Gain58 : Gain  Gain=10
  Gain6 : Gain  Gain=-5
  Gain60 : Gain  Gain=7
  Gain61 : Gain  Gain=9
  Gain62 : Gain  Gain=-12
  Gain63 : Gain  Gain=-24
  Gain64 : Gain  Gain=-15
  Gain65 : Gain  Gain=-21
  Gain66 : Gain  Gain=-20
  Gain67 : Gain  Gain=-18
  Gain7 : Gain  Gain=4
  Gain8 : Gain  Gain=4
  Idq_Shunt_Scope : Scope  NumInputPorts=8
  Idq_Shunt_Scope_f : Scope  NumInputPorts=8
  Selector : Selector  InputPortWidth=3  IndexOptions=Index vector (dialog)  Indices=[1 2]  OutputSizes=1
  Selector1 : Selector  InputPortWidth=3  IndexOptions=Index vector (dialog)  Indices=[3]  OutputSizes=1
  Shunt_dekomp_INetz_dqplus1_Scope : Scope  NumInputPorts=2
  Shunt_dekomp_INetz_dqplus2_Scope : Scope  NumInputPorts=2
  Shunt_dekomp_INetz_dqplus3_Scope : Scope  NumInputPorts=2
  Shunt_dekomp_INetz_dqplus4_Scope : Scope  NumInputPorts=2
  Tdq+1_1 : Subsystem
  Tdq+1_2 : Subsystem
  Tdq+1_3 : Subsystem
  Tdq+1_4 : Subsystem
  Tdq+1_5 : Subsystem
  Tdq+1_6 : Subsystem
  Tdq+1_7 : Subsystem
  Tdq+1_8 : Subsystem
  Unit Delay{1..8} (8 alike) : UnitDelay  SampleTime=-1  HasFrameUpgradeWarning=on
  Out5 : Outport
  wires:
  [null] -> Bus Creator/17  "null"
  [idqp19_f] -> Bus Creator/16
  [idqg8_f] -> Bus Creator/15
  [idqp7_f] -> Bus Creator/14
  [idqg5_f] -> Bus Creator/13
  [idqp4_f] -> Bus Creator/12
  [idqg2_f] -> Bus Creator/11
  [idqp1_f] -> Bus Creator/9
  [idqg1_f] -> Bus Creator/10
  [idqp19] -> Bus Creator/8
  [idqg8] -> Bus Creator/7
  [idqp7] -> Bus Creator/6
  [idqg5] -> Bus Creator/5
  [idqp4] -> Bus Creator/4
  [idqg2] -> Bus Creator/3
  [idqg1] -> Bus Creator/2
  [idqp1] -> Bus Creator/1
  [idqp19] -> Idq_Shunt_Scope/8
  [idqg8] -> Idq_Shunt_Scope/7
  [idqp7] -> Idq_Shunt_Scope/6
  [idqg5] -> Idq_Shunt_Scope/5
  [idqp4] -> Idq_Shunt_Scope/4
  [idqg2] -> Idq_Shunt_Scope/3
  [idqg1] -> Idq_Shunt_Scope/2
  [idqp1] -> Idq_Shunt_Scope/1
  Entkopplungszelle45/1(Out2) -> Unit Delay8/1
  First-Order Filter8/1 -> Gain71/1  "idqp19_f"
  Gain71/1 -> [idqp19_f]  "idqp19_f"
  Unit Delay8/1 -> First-Order Filter8/1, [idqp19]  "idqp19"
  Unit Delay7/1 -> [idqg8], First-Order Filter7/1  "idqg8"
  Gain70/1 -> [idqg8_f]  "idqg8_f"
  First-Order Filter7/1 -> Gain70/1  "idqg8_f"
  Unit Delay6/1 -> [idqg2], First-Order Filter6/1  "idqg2"
  Gain69/1 -> [idqg2_f]  "idqg2_f"
  First-Order Filter6/1 -> Gain69/1  "idqg2_f"
  Unit Delay5/1 -> [idqp7], First-Order Filter5/1  "idqp7"
  Gain68/1 -> [idqp7_f]  "idqp7_f"
  First-Order Filter5/1 -> Gain68/1  "idqp7_f"
  [idqp19_f] -> Entkopplungszelle56/3(In1)
  Gain67/1 -> Entkopplungszelle56/2(In4)
  [theta] -> Gain67/1
  Entkopplungszelle50/1(Out2) -> Entkopplungszelle56/1(In3)
  Entkopplungszelle49/1(Out2) -> Entkopplungszelle55/1(In3)
  [theta] -> Gain66/1
  Gain66/1 -> Entkopplungszelle55/2(In4)
  [idqp19_f] -> Entkopplungszelle55/3(In1)
  [idqp19_f] -> Entkopplungszelle54/3(In1)
  Gain65/1 -> Entkopplungszelle54/2(In4)
  [theta] -> Gain65/1
  Entkopplungszelle48/1(Out2) -> Entkopplungszelle54/1(In3)
  Entkopplungszelle47/1(Out2) -> Entkopplungszelle53/1(In3)
  [theta] -> Gain64/1
  Gain64/1 -> Entkopplungszelle53/2(In4)
  [idqp19_f] -> Entkopplungszelle53/3(In1)
  Entkopplungszelle46/1(Out2) -> Entkopplungszelle52/1(In3)
  [idqp19_f] -> Entkopplungszelle52/3(In1)
  Gain63/1 -> Entkopplungszelle52/2(In4)
  [theta] -> Gain63/1
  [theta] -> Gain62/1
  Gain62/1 -> Entkopplungszelle51/2(In4)
  [idqp19_f] -> Entkopplungszelle51/3(In1)
  Entkopplungszelle41/1(Out2) -> Entkopplungszelle51/1(In3)
  Entkopplungszelle37/1(Out2) -> Entkopplungszelle50/1(In3)
  [theta] -> Gain61/1
  Gain61/1 -> Entkopplungszelle50/2(In4)
  [idqg8_f] -> Entkopplungszelle50/3(In1)
  [idqg8_f] -> Entkopplungszelle49/3(In1)
  Gain60/1 -> Entkopplungszelle49/2(In4)
  [theta] -> Gain60/1
  Entkopplungszelle38/1(Out2) -> Entkopplungszelle49/1(In3)
  Entkopplungszelle39/1(Out2) -> Entkopplungszelle48/1(In3)
  [theta] -> Gain59/1
  Gain59/1 -> Entkopplungszelle48/2(In4)
  [idqg8_f] -> Entkopplungszelle48/3(In1)
  Entkopplungszelle40/1(Out2) -> Entkopplungszelle47/1(In3)
  [idqg8_f] -> Entkopplungszelle47/3(In1)
  Gain58/1 -> Entkopplungszelle47/2(In4)
  [theta] -> Gain58/1
  [theta] -> Gain57/1
  Gain57/1 -> Entkopplungszelle46/2(In4)
  [idqg8_f] -> Entkopplungszelle46/3(In1)
  Entkopplungszelle36/1(Out2) -> Entkopplungszelle46/1(In3)
  Entkopplungszelle43/1(Out2) -> Entkopplungszelle45/1(In3)
  [idqg8_f] -> Entkopplungszelle45/3(In1)
  Gain56/1 -> Entkopplungszelle45/2(In4)
  [theta] -> Gain56/1
  Entkopplungszelle42/1(Out2) -> Entkopplungszelle44/1(In3)
  [idqp19_f] -> Entkopplungszelle44/3(In1)
  Gain55/1 -> Entkopplungszelle44/2(In4)
  [theta] -> Gain55/1
  [idqp7_f] -> Entkopplungszelle43/3(In1)
  Gain54/1 -> Entkopplungszelle43/2(In4)
  [theta] -> Gain54/1
  Entkopplungszelle35/1(Out2) -> Entkopplungszelle43/1(In3)
  Entkopplungszelle34/1(Out2) -> Entkopplungszelle42/1(In3)
  [theta] -> Gain53/1
  Gain53/1 -> Entkopplungszelle42/2(In4)
  [idqp7_f] -> Entkopplungszelle42/3(In1)
  [theta] -> Gain52/1
  Gain52/1 -> Entkopplungszelle41/2(In4)
  [idqg8_f] -> Entkopplungszelle41/3(In1)
  Entkopplungszelle33/1(Out2) -> Entkopplungszelle41/1(In3)
  Entkopplungszelle9/1(Out2) -> Entkopplungszelle40/1(In3)
  [idqp7_f] -> Entkopplungszelle40/3(In1)
  Gain51/1 -> Entkopplungszelle40/2(In4)
  [theta] -> Gain51/1
  Entkopplungszelle29/1(Out2) -> Entkopplungszelle39/1(In3)
  [theta] -> Gain50/1
  Gain50/1 -> Entkopplungszelle39/2(In4)
  [idqp7_f] -> Entkopplungszelle39/3(In1)
  [idqp7_f] -> Entkopplungszelle38/3(In1)
  Gain49/1 -> Entkopplungszelle38/2(In4)
  [theta] -> Gain49/1
  Entkopplungszelle6/1(Out2) -> Entkopplungszelle38/1(In3)
  Entkopplungszelle4/1(Out2) -> Entkopplungszelle37/1(In3)
  [theta] -> Gain48/1
  Gain48/1 -> Entkopplungszelle37/2(In4)
  [idqp7_f] -> Entkopplungszelle37/3(In1)
  [idqp7_f] -> Entkopplungszelle36/3(In1)
  Gain47/1 -> Entkopplungszelle36/2(In4)
  [theta] -> Gain47/1
  Entkopplungszelle12/1(Out2) -> Entkopplungszelle36/1(In3)
  Entkopplungszelle32/1(Out2) -> Entkopplungszelle35/1(In3)
  [idqg5_f] -> Entkopplungszelle35/3(In1)
  Gain46/1 -> Entkopplungszelle35/2(In4)
  [theta] -> Gain46/1
  Entkopplungszelle31/1(Out2) -> Entkopplungszelle34/1(In3)
  [theta] -> Gain45/1
  Gain45/1 -> Entkopplungszelle34/2(In4)
  [idqg5_f] -> Entkopplungszelle34/3(In1)
  [idqg5_f] -> Entkopplungszelle33/3(In1)
  Gain44/1 -> Entkopplungszelle33/2(In4)
  [theta] -> Gain44/1
  Entkopplungszelle30/1(Out2) -> Entkopplungszelle33/1(In3)
  [idqp4_f] -> Entkopplungszelle32/3(In1)
  Gain43/1 -> Entkopplungszelle32/2(In4)
  [theta] -> Gain43/1
  Entkopplungszelle27/1(Out2) -> Entkopplungszelle32/1(In3)
  Entkopplungszelle26/1(Out2) -> Entkopplungszelle31/1(In3)
  [theta] -> Gain42/1
  Gain42/1 -> Entkopplungszelle31/2(In4)
  [idqp4_f] -> Entkopplungszelle31/3(In1)
  [idqp4_f] -> Entkopplungszelle30/3(In1)
  Gain41/1 -> Entkopplungszelle30/2(In4)
  [theta] -> Gain41/1
  Entkopplungszelle25/1(Out2) -> Entkopplungszelle30/1(In3)
  Entkopplungszelle24/1(Out2) -> Entkopplungszelle12/1(In3)
  Entkopplungszelle23/1(Out2) -> Entkopplungszelle9/1(In3)
  [theta] -> Gain39/1
  [idqg5_f] -> Entkopplungszelle29/3(In1)
  [idqp4_f] -> Entkopplungszelle28/3(In1)
  Gain40/1 -> Entkopplungszelle29/2(In4)
  Gain39/1 -> Entkopplungszelle28/2(In4)
  [theta] -> Gain40/1
  Entkopplungszelle28/1(Out2) -> Entkopplungszelle29/1(In3)
  Entkopplungszelle17/1(Out2) -> Entkopplungszelle28/1(In3)
  [idqg2_f] -> Entkopplungszelle27/3(In1)
  Gain38/1 -> Entkopplungszelle27/2(In4)
  [theta] -> Gain38/1
  Entkopplungszelle20/1(Out2) -> Entkopplungszelle27/1(In3)
  Entkopplungszelle19/1(Out2) -> Entkopplungszelle26/1(In3)
  [theta] -> Gain37/1
  Gain37/1 -> Entkopplungszelle26/2(In4)
  [idqg2_f] -> Entkopplungszelle26/3(In1)
  Entkopplungszelle18/1(Out2) -> Entkopplungszelle25/1(In3)
  [idqg2_f] -> Entkopplungszelle25/3(In1)
  Gain36/1 -> Entkopplungszelle25/2(In4)
  [theta] -> Gain36/1
  [theta] -> Gain35/1
  Gain35/1 -> Entkopplungszelle24/2(In4)
  [idqg2_f] -> Entkopplungszelle24/3(In1)
  Entkopplungszelle10/1(Out2) -> Entkopplungszelle24/1(In3)
  Entkopplungszelle7/1(Out2) -> Entkopplungszelle23/1(In3)
  [idqg2_f] -> Entkopplungszelle23/3(In1)
  Gain34/1 -> Entkopplungszelle23/2(In4)
  [theta] -> Gain34/1
  Entkopplungszelle22/1(Out2) -> Entkopplungszelle3/1(In3)
  [theta] -> Gain33/1
  Gain33/1 -> Entkopplungszelle22/2(In4)
  [idqg2_f] -> Entkopplungszelle22/3(In1)
  Entkopplungszelle5/1(Out2) -> Entkopplungszelle22/1(In3)
  Entkopplungszelle21/1(Out2) -> Entkopplungszelle1/1(In3)
  Entkopplungszelle2/1(Out2) -> Entkopplungszelle21/1(In3)
  [idqg2_f] -> Entkopplungszelle21/3(In1)
  Gain32/1 -> Entkopplungszelle21/2(In4)
  [theta] -> Gain32/1
  Gain31/1 -> Entkopplungszelle20/2(In4)
  Entkopplungszelle16/1(Out2) -> Entkopplungszelle20/1(In3)
  [idqg1_f] -> Entkopplungszelle20/3(In1)
  [theta] -> Gain31/1
  [theta] -> Gain30/1
  [idqg1_f] -> Entkopplungszelle19/3(In1)
  Entkopplungszelle15/1(Out2) -> Entkopplungszelle19/1(In3)
  Gain30/1 -> Entkopplungszelle19/2(In4)
  Gain29/1 -> Entkopplungszelle18/2(In4)
  Entkopplungszelle14/1(Out2) -> Entkopplungszelle18/1(In3)
  [idqg1_f] -> Entkopplungszelle18/3(In1)
  [theta] -> Gain29/1
  [theta] -> Gain28/1
  [idqg1_f] -> Entkopplungszelle17/3(In1)
  Entkopplungszelle13/1(Out2) -> Entkopplungszelle17/1(In3)
  Gain28/1 -> Entkopplungszelle17/2(In4)
  [idqp1_f] -> Entkopplungszelle16/3(In1)
  [idqp1_f] -> Entkopplungszelle15/3(In1)
  [idqp1_f] -> Entkopplungszelle14/3(In1)
  Gain27/1 -> Entkopplungszelle16/2(In4)
  Tdq+1_8/1(Out1) -> Entkopplungszelle16/1(In3)
  [theta] -> Gain27/1
  [theta] -> Gain26/1
  Tdq+1_7/1(Out1) -> Entkopplungszelle15/1(In3)
  Gain26/1 -> Entkopplungszelle15/2(In4)
  Gain25/1 -> Entkopplungszelle14/2(In4)
  Tdq+1_6/1(Out1) -> Entkopplungszelle14/1(In3)
  [theta] -> Gain25/1
  Tdq+1_5/1(Out1) -> Entkopplungszelle13/1(In3)
  [theta] -> Gain24/1
  Gain24/1 -> Entkopplungszelle13/2(In4)
  [idqp1_f] -> Entkopplungszelle13/3(In1)
  [theta] -> Gain23/1
  Gain23/1 -> Tdq+1_8/2(In2)
  [iab] -> Tdq+1_8/1(In1)
  [iab] -> Tdq+1_7/1(In1)
  Gain22/1 -> Tdq+1_7/2(In2)
  [theta] -> Gain22/1
  [theta] -> Gain21/1
  Gain21/1 -> Tdq+1_6/2(In2)
  [iab] -> Tdq+1_6/1(In1)
  Gain20/1 -> Tdq+1_5/2(In2)
  [iab] -> Tdq+1_5/1(In1)
  [theta] -> Gain20/1
  First-Order Filter4/1 -> Gain19/1  "idqg5_f"
  First-Order Filter3/1 -> Gain18/1  "idqp4_f"
  First-Order Filter2/1 -> Gain17/1  "idqg1_f"
  First-Order Filter1/1 -> Gain16/1  "idqp1_f"
  Entkopplungszelle8/1(Out2) -> Entkopplungszelle7/1(In3)
  Entkopplungszelle1/1(Out2) -> Entkopplungszelle4/1(In3)
  Entkopplungszelle3/1(Out2) -> Entkopplungszelle6/1(In3)
  Entkopplungszelle11/1(Out2) -> Entkopplungszelle10/1(In3)
  Gain19/1 -> [idqg5_f]  "idqg5_f"
  Gain18/1 -> [idqp4_f]  "idqp4_f"
  Gain17/1 -> [idqg1_f]  "idqg1_f"
  Gain16/1 -> [idqp1_f]  "idqp1_f"
  Bus Creator/1 -> Out5/1  "idq_B"
  [idqp1_f] -> Entkopplungszelle11/3(In1)
  [theta] -> Gain15/1
  Gain14/1 -> Entkopplungszelle10/2(In4)
  Unit Delay4/1 -> First-Order Filter4/1, [idqg5]  "idqg5"
  Gain15/1 -> Entkopplungszelle12/2(In4)
  Gain13/1 -> Entkopplungszelle11/2(In4)
  Tdq+1_4/1(Out1) -> Shunt_dekomp_INetz_dqplus4_Scope/2, Entkopplungszelle11/1(In3)
  [theta] -> Gain13/1
  [iab] -> Tdq+1_4/1(In1), Shunt_dekomp_INetz_dqplus4_Scope/1
  Gain12/1 -> Tdq+1_4/2(In2)
  [theta] -> Gain12/1
  [idqg1_f] -> Entkopplungszelle10/3(In1)
  [idqp4_f] -> Entkopplungszelle12/3(In1)
  [theta] -> Gain14/1
  [idqp1_f] -> Entkopplungszelle8/3(In1)
  [theta] -> Gain11/1
  Gain10/1 -> Entkopplungszelle7/2(In4)
  Unit Delay3/1 -> First-Order Filter3/1, [idqp4]  "idqp4"
  Gain11/1 -> Entkopplungszelle9/2(In4)
  Gain9/1 -> Entkopplungszelle8/2(In4)
  Tdq+1_3/1(Out1) -> Shunt_dekomp_INetz_dqplus3_Scope/2, Entkopplungszelle8/1(In3)
  [theta] -> Gain9/1
  [iab] -> Tdq+1_3/1(In1), Shunt_dekomp_INetz_dqplus3_Scope/1
  Gain8/1 -> Tdq+1_3/2(In2)
  [theta] -> Gain8/1
  [idqg1_f] -> Entkopplungszelle7/3(In1)
  [idqg5_f] -> Entkopplungszelle9/3(In1)
  [theta] -> Gain10/1
  [idqp1_f] -> Entkopplungszelle5/3(In1)
  [theta] -> Gain7/1
  Gain6/1 -> Entkopplungszelle3/2(In4)
  Unit Delay2/1 -> First-Order Filter2/1, [idqg1]  "idqg1"
  Gain7/1 -> Entkopplungszelle6/2(In4)
  Gain5/1 -> Entkopplungszelle5/2(In4)
  Tdq+1_2/1(Out1) -> Shunt_dekomp_INetz_dqplus2_Scope/2, Entkopplungszelle5/1(In3)
  [theta] -> Gain5/1
  [iab] -> Tdq+1_2/1(In1), Shunt_dekomp_INetz_dqplus2_Scope/1
  Gain4/1 -> Tdq+1_2/2(In2)
  [theta] -> Gain4/1
  [idqp4_f] -> Entkopplungszelle3/3(In1)
  [idqg5_f] -> Entkopplungszelle6/3(In1)
  [theta] -> Gain6/1
  Gain3/1 -> Entkopplungszelle4/2(In4)
  Gain2/1 -> Entkopplungszelle1/2(In4)
  [theta] -> Gain2/1
  Gain1/1 -> Entkopplungszelle2/2(In4)
  Unit Delay1/1 -> First-Order Filter1/1, [idqp1]  "idqp1"
  [idqg5_f] -> Entkopplungszelle4/3(In1)
  [theta] -> Gain3/1
  [idqp4_f] -> Entkopplungszelle1/3(In1)
  Selector1/1 -> [null]
  Selector/1 -> [iab]
  Gain/1 -> Tdq+1_1/2(In2)
  [theta] -> Gain/1
  In1/1 -> [theta]  "phipll"
  [Igabc] -> Clarke Transform1/1
  Tdq+1_1/1(Out1) -> Shunt_dekomp_INetz_dqplus1_Scope/2, Entkopplungszelle2/1(In3)
  [idqg1_f] -> Entkopplungszelle2/3(In1)
  [iab] -> Tdq+1_1/1(In1), Shunt_dekomp_INetz_dqplus1_Scope/1
  In2/1 -> [Igabc]  "Iabc"
  [theta] -> Gain1/1
  Clarke Transform1/1 -> Selector1/1, Selector/1
  [idqp1_f] -> Idq_Shunt_Scope_f/1
  [idqg1_f] -> Idq_Shunt_Scope_f/2
  [idqg2_f] -> Idq_Shunt_Scope_f/3
  [idqp4_f] -> Idq_Shunt_Scope_f/4
  [idqg5_f] -> Idq_Shunt_Scope_f/5
  [idqp7_f] -> Idq_Shunt_Scope_f/6
  [idqg8_f] -> Idq_Shunt_Scope_f/7
  [idqp19_f] -> Idq_Shunt_Scope_f/8
  Entkopplungszelle44/1(Out2) -> Unit Delay7/1
  Entkopplungszelle51/1(Out2) -> Unit Delay5/1
  Entkopplungszelle52/1(Out2) -> Unit Delay4/1
  Entkopplungszelle53/1(Out2) -> Unit Delay3/1
  Entkopplungszelle54/1(Out2) -> Unit Delay6/1
  Entkopplungszelle55/1(Out2) -> Unit Delay2/1
  Entkopplungszelle56/1(Out2) -> Unit Delay1/1
